simulink model "FaultModel (1)"  (R2018b)
settings: Solver=VariableStepAuto  StartTime=0.0  StopTime=0.05  RelTol=1e-3
undefined symbols (not defined in the file or in its folder): D1, Delta
libraries: powerlib x316
(part 1 of 4)
settings Model: Creator=DELL  LastModifiedBy=DELL
settings DataIOCC: ReturnWorkspaceOutputs=on
settings DebuggingCC: UnconnectedInputMsg=none  UnconnectedOutputMsg=none  UnconnectedLineMsg=none  SFMachineParentedDataDiag=error
settings ModelReferenceCC: EnableRefExpFcnMdlSchedulingChecks=off
settings RTWCC: Description=Generic Real-Time Target

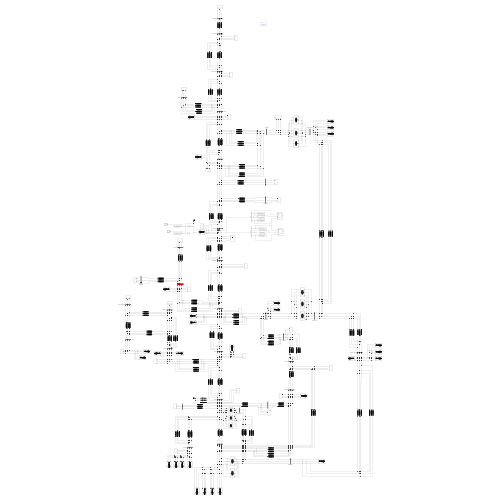
[thumbnail: Simulink's stored preview of the top-level diagram]
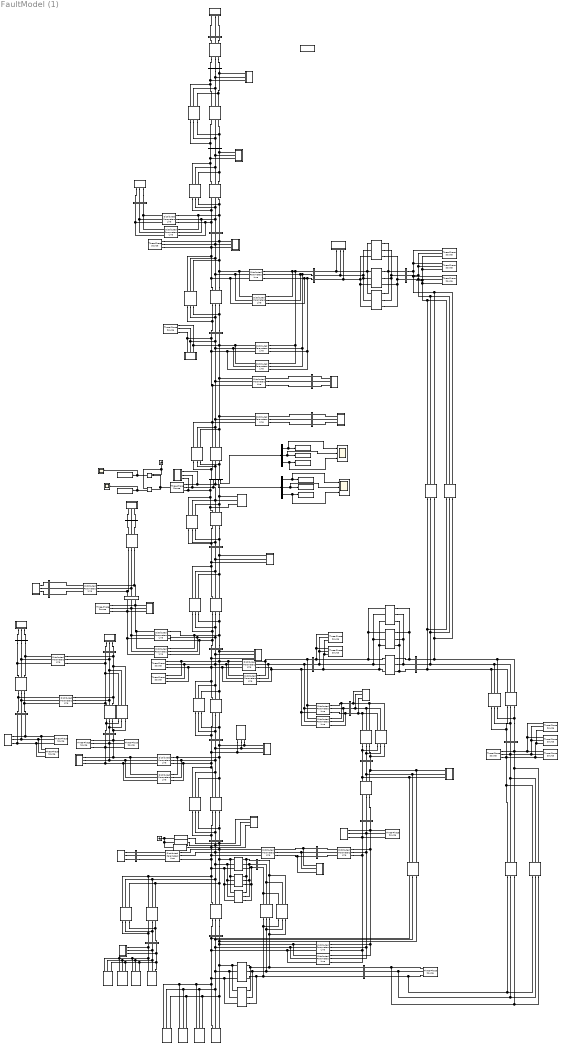
== system FaultModel (1) ==
  Amnura : powerlib/Measurements/Three-Phase V-I Measurement  VoltageMeasurement=no  SetLabelV=off  LabelV=Vabc  Vpu=off  VpuLL=off  CurrentMeasurement=no  SetLabelI=off  LabelI=Iabc  Ipu=off  Pbase=100e6  Vbase=500e3  OutputType=Complex  PhasorSimulation=off  PSBequivalent=0
  Baghabari : powerlib/Measurements/Three-Phase V-I Measurement  VoltageMeasurement=no  SetLabelV=off  LabelV=Vabc  Vpu=off  VpuLL=off  CurrentMeasurement=no  SetLabelI=off  LabelI=Iabc  Ipu=off  Pbase=100e6  Vbase=500e3  OutputType=Complex  PhasorSimulation=off  PSBequivalent=0
  Baghabari PP : powerlib/Measurements/Three-Phase V-I Measurement  VoltageMeasurement=no  SetLabelV=off  LabelV=Vabc  Vpu=off  VpuLL=off  CurrentMeasurement=no  SetLabelI=off  LabelI=Iabc  Ipu=off  Pbase=100e6  Vbase=500e3  OutputType=Complex  PhasorSimulation=off  PSBequivalent=0
  Barapukuria : powerlib/Measurements/Three-Phase V-I Measurement  VoltageMeasurement=no  SetLabelV=off  LabelV=Vabc  Vpu=off  VpuLL=off  CurrentMeasurement=no  SetLabelI=off  LabelI=Iabc  Ipu=off  Pbase=100e6  Vbase=500e3  OutputType=Complex  PhasorSimulation=off  PSBequivalent=0
  Barapukuria PP : powerlib/Measurements/Three-Phase V-I Measurement  VoltageMeasurement=no  SetLabelV=off  LabelV=Vabc  Vpu=off  VpuLL=off  CurrentMeasurement=no  SetLabelI=off  LabelI=Iabc  Ipu=off  Pbase=100e6  Vbase=500e3  OutputType=Complex  PhasorSimulation=off  PSBequivalent=0
  Bheramara : powerlib/Measurements/Three-Phase V-I Measurement  VoltageMeasurement=no  SetLabelV=off  LabelV=Vabc  Vpu=off  VpuLL=off  CurrentMeasurement=no  SetLabelI=off  LabelI=Iabc  Ipu=off  Pbase=100e6  Vbase=500e3  OutputType=Complex  PhasorSimulation=off  PSBequivalent=0
  Bogura : powerlib/Measurements/Three-Phase V-I Measurement  VoltageMeasurement=no  SetLabelV=off  LabelV=Vabc  Vpu=off  VpuLL=off  CurrentMeasurement=no  SetLabelI=off  LabelI=Iabc  Ipu=off  Pbase=100e6  Vbase=500e3  OutputType=Complex  PhasorSimulation=off  PSBequivalent=0
  Bogura New : powerlib/Measurements/Three-Phase V-I Measurement  VoltageMeasurement=no  SetLabelV=off  LabelV=Vabc  Vpu=off  VpuLL=off  CurrentMeasurement=no  SetLabelI=off  LabelI=Iabc  Ipu=off  Pbase=100e6  Vbase=500e3  OutputType=Complex  PhasorSimulation=off  PSBequivalent=0
  Bogura New PP : powerlib/Measurements/Three-Phase V-I Measurement  VoltageMeasurement=no  SetLabelV=off  LabelV=Vabc  Vpu=off  VpuLL=off  CurrentMeasurement=no  SetLabelI=off  LabelI=Iabc  Ipu=off  Pbase=100e6  Vbase=500e3  OutputType=Complex  PhasorSimulation=off  PSBequivalent=0
  Chapai Nawabganj : powerlib/Measurements/Three-Phase V-I Measurement  VoltageMeasurement=no  SetLabelV=off  LabelV=Vabc  Vpu=off  VpuLL=off  CurrentMeasurement=no  SetLabelI=off  LabelI=Iabc  Ipu=off  Pbase=100e6  Vbase=500e3  OutputType=Complex  PhasorSimulation=off  PSBequivalent=0
  Current Measurement : powerlib/Measurements/Current Measurement  PhasorSimulation=off  OutputType=Complex  PSBequivalent=0
  Demux : Demux  Outputs=3
  Demux1 : Demux  Outputs=3
  Distributed Parameters Line : powerlib/Elements/Distributed Parameters Line  Phases=3  Length=45  Frequency=50  Resistance=[0.01273 0.3864]  Inductance="[0.9337e-3  4.1264e-3]"  Capacitance=[12.74e-9 7.751e-9]  x1=[0 0 0 0; 0.0001244 0 0 0; 0.0002488 0 0 0; 0.0003733 0 0 0; 0.0004977 0 0 0; 0.0006221 0 0 0]  x2=[0 0 0 0; 0.0001244 0 0 0; 0.0002488 0 0 0; 0.0003733 0 0 0; 0.0004977 0 0 0; 0.0006221 0 0 0]  x3=[0 0 0 0; 0.0001244 0 0 0; 0.0002488 0 0 0; 0.0003733 0 0 0; 0.0004977 0 0 0; 0.0006221 0 0 0]  x4=[0 0 0 0; 0.0001244 0 0 0; 0.0002488 0 0 0; 0.0003733 0 0 0; 0.0004977 0 0 0; 0.0006221 0 0 0]  x5=0  V1=ones(3,3)  V2=ones(3,3)  I1=ones(3,3)  I2=ones(3,3)  nHarmo=1  Measurements=None  Decoupling=off  VsMag0=0  VrMag0=0  VsAngle0=0  VrAngle0=0  IsMag0=0  IrMag0=0  IsAngle0=0  IrAngle0=0
  Distributed Parameters Line1 : powerlib/Elements/Distributed Parameters Line  Phases=3  Length=45  Frequency=50  Resistance=[0.01273 0.3864]  Inductance="[0.9337e-3  4.1264e-3]"  Capacitance=[12.74e-9 7.751e-9]  x1=[0 0 0 0; 0.0001244 0 0 0; 0.0002488 0 0 0; 0.0003733 0 0 0; 0.0004977 0 0 0; 0.0006221 0 0 0]  x2=[0 0 0 0; 0.0001244 0 0 0; 0.0002488 0 0 0; 0.0003733 0 0 0; 0.0004977 0 0 0; 0.0006221 0 0 0]  x3=[0 0 0 0; 0.0001244 0 0 0; 0.0002488 0 0 0; 0.0003733 0 0 0; 0.0004977 0 0 0; 0.0006221 0 0 0]  x4=[0 0 0 0; 0.0001244 0 0 0; 0.0002488 0 0 0; 0.0003733 0 0 0; 0.0004977 0 0 0; 0.0006221 0 0 0]  x5=0  V1=ones(3,3)  V2=ones(3,3)  I1=ones(3,3)  I2=ones(3,3)  nHarmo=1  Measurements=None  Decoupling=off  VsMag0=0  VrMag0=0  VsAngle0=0  VrAngle0=0  IsMag0=0  IrMag0=0  IsAngle0=0  IrAngle0=0
  Distributed Parameters Line{9..10,44..45} (4 alike) : powerlib/Elements/Distributed Parameters Line  Phases=3  Length=36  Frequency=50  Resistance=[0.01273 0.3864]  Inductance="[0.9337e-3  4.1264e-3]"  Capacitance=[12.74e-9 7.751e-9]  x1=[0 0 0 0; 0.0001244 0 0 0; 0.0002488 0 0 0; 0.0003733 0 0 0; 0.0004977 0 0 0; 0.0006221 0 0 0]  x2=[0 0 0 0; 0.0001244 0 0 0; 0.0002488 0 0 0; 0.0003733 0 0 0; 0.0004977 0 0 0; 0.0006221 0 0 0]  x3=[0 0 0 0; 0.0001244 0 0 0; 0.0002488 0 0 0; 0.0003733 0 0 0; 0.0004977 0 0 0; 0.0006221 0 0 0]  x4=[0 0 0 0; 0.0001244 0 0 0; 0.0002488 0 0 0; 0.0003733 0 0 0; 0.0004977 0 0 0; 0.0006221 0 0 0]  x5=0  V1=ones(3,3)  V2=ones(3,3)  I1=ones(3,3)  I2=ones(3,3)  nHarmo=1  Measurements=None  Decoupling=off  VsMag0=0  VrMag0=0  VsAngle0=0  VrAngle0=0  IsMag0=0  IrMag0=0  IsAngle0=0  IrAngle0=0
  Distributed Parameters Line{11..12,29..30} (4 alike) : powerlib/Elements/Distributed Parameters Line  Phases=3  Length=42  Frequency=50  Resistance=[0.01273 0.3864]  Inductance="[0.9337e-3  4.1264e-3]"  Capacitance=[12.74e-9 7.751e-9]  x1=[0 0 0 0; 0.0001244 0 0 0; 0.0002488 0 0 0; 0.0003733 0 0 0; 0.0004977 0 0 0; 0.0006221 0 0 0]  x2=[0 0 0 0; 0.0001244 0 0 0; 0.0002488 0 0 0; 0.0003733 0 0 0; 0.0004977 0 0 0; 0.0006221 0 0 0]  x3=[0 0 0 0; 0.0001244 0 0 0; 0.0002488 0 0 0; 0.0003733 0 0 0; 0.0004977 0 0 0; 0.0006221 0 0 0]  x4=[0 0 0 0; 0.0001244 0 0 0; 0.0002488 0 0 0; 0.0003733 0 0 0; 0.0004977 0 0 0; 0.0006221 0 0 0]  x5=0  V1=ones(3,3)  V2=ones(3,3)  I1=ones(3,3)  I2=ones(3,3)  nHarmo=1  Measurements=None  Decoupling=off  VsMag0=0  VrMag0=0  VsAngle0=0  VrAngle0=0  IsMag0=0  IrMag0=0  IsAngle0=0  IrAngle0=0
  Distributed Parameters Line13 : powerlib/Elements/Distributed Parameters Line  Phases=3  Length=40.95  Frequency=50  Resistance=[0.01273 0.3864]  Inductance="[0.9337e-3  4.1264e-3]"  Capacitance=[12.74e-9 7.751e-9]  x1=[0 0 0 0; 0.0001244 0 0 0; 0.0002488 0 0 0; 0.0003733 0 0 0; 0.0004977 0 0 0; 0.0006221 0 0 0]  x2=[0 0 0 0; 0.0001244 0 0 0; 0.0002488 0 0 0; 0.0003733 0 0 0; 0.0004977 0 0 0; 0.0006221 0 0 0]  x3=[0 0 0 0; 0.0001244 0 0 0; 0.0002488 0 0 0; 0.0003733 0 0 0; 0.0004977 0 0 0; 0.0006221 0 0 0]  x4=[0 0 0 0; 0.0001244 0 0 0; 0.0002488 0 0 0; 0.0003733 0 0 0; 0.0004977 0 0 0; 0.0006221 0 0 0]  x5=0  V1=ones(3,3)  V2=ones(3,3)  I1=ones(3,3)  I2=ones(3,3)  nHarmo=1  Measurements=None  Decoupling=off  VsMag0=0  VrMag0=0  VsAngle0=0  VrAngle0=0  IsMag0=0  IrMag0=0  IsAngle0=0  IrAngle0=0
  Distributed Parameters Line14 : powerlib/Elements/Distributed Parameters Line  Phases=3  Length=38  Frequency=50  Resistance=[0.01273 0.3864]  Inductance="[0.9337e-3  4.1264e-3]"  Capacitance=[12.74e-9 7.751e-9]  x1=[0 0 0 0; 0.0001244 0 0 0; 0.0002488 0 0 0; 0.0003733 0 0 0; 0.0004977 0 0 0; 0.0006221 0 0 0]  x2=[0 0 0 0; 0.0001244 0 0 0; 0.0002488 0 0 0; 0.0003733 0 0 0; 0.0004977 0 0 0; 0.0006221 0 0 0]  x3=[0 0 0 0; 0.0001244 0 0 0; 0.0002488 0 0 0; 0.0003733 0 0 0; 0.0004977 0 0 0; 0.0006221 0 0 0]  x4=[0 0 0 0; 0.0001244 0 0 0; 0.0002488 0 0 0; 0.0003733 0 0 0; 0.0004977 0 0 0; 0.0006221 0 0 0]  x5=0  V1=ones(3,3)  V2=ones(3,3)  I1=ones(3,3)  I2=ones(3,3)  nHarmo=1  Measurements=None  Decoupling=off  VsMag0=0  VrMag0=0  VsAngle0=0  VrAngle0=0  IsMag0=0  IrMag0=0  IsAngle0=0  IrAngle0=0
  Distributed Parameters Line15 : powerlib/Elements/Distributed Parameters Line  Phases=3  Length=52  Frequency=50  Resistance=[0.01273 0.3864]  Inductance="[0.9337e-3  4.1264e-3]"  Capacitance=[12.74e-9 7.751e-9]  x1=[0 0 0 0; 0.0001244 0 0 0; 0.0002488 0 0 0; 0.0003733 0 0 0; 0.0004977 0 0 0; 0.0006221 0 0 0]  x2=[0 0 0 0; 0.0001244 0 0 0; 0.0002488 0 0 0; 0.0003733 0 0 0; 0.0004977 0 0 0; 0.0006221 0 0 0]  x3=[0 0 0 0; 0.0001244 0 0 0; 0.0002488 0 0 0; 0.0003733 0 0 0; 0.0004977 0 0 0; 0.0006221 0 0 0]  x4=[0 0 0 0; 0.0001244 0 0 0; 0.0002488 0 0 0; 0.0003733 0 0 0; 0.0004977 0 0 0; 0.0006221 0 0 0]  x5=0  V1=ones(3,3)  V2=ones(3,3)  I1=ones(3,3)  I2=ones(3,3)  nHarmo=1  Measurements=None  Decoupling=off  VsMag0=0  VrMag0=0  VsAngle0=0  VrAngle0=0  IsMag0=0  IrMag0=0  IsAngle0=0  IrAngle0=0
  Distributed Parameters Line16 : powerlib/Elements/Distributed Parameters Line  Phases=3  Length=52  Frequency=50  Resistance=[0.01273 0.3864]  Inductance="[0.9337e-3  4.1264e-3]"  Capacitance=[12.74e-9 7.751e-9]  x1=[0 0 0 0; 0.0001244 0 0 0; 0.0002488 0 0 0; 0.0003733 0 0 0; 0.0004977 0 0 0; 0.0006221 0 0 0]  x2=[0 0 0 0; 0.0001244 0 0 0; 0.0002488 0 0 0; 0.0003733 0 0 0; 0.0004977 0 0 0; 0.0006221 0 0 0]  x3=[0 0 0 0; 0.0001244 0 0 0; 0.0002488 0 0 0; 0.0003733 0 0 0; 0.0004977 0 0 0; 0.0006221 0 0 0]  x4=[0 0 0 0; 0.0001244 0 0 0; 0.0002488 0 0 0; 0.0003733 0 0 0; 0.0004977 0 0 0; 0.0006221 0 0 0]  x5=0  V1=ones(3,3)  V2=ones(3,3)  I1=ones(3,3)  I2=ones(3,3)  nHarmo=1  Measurements=None  Decoupling=off  VsMag0=0  VrMag0=0  VsAngle0=0  VrAngle0=0  IsMag0=0  IrMag0=0  IsAngle0=0  IrAngle0=0
  Distributed Parameters Line17 : powerlib/Elements/Distributed Parameters Line  Phases=3  Length=0.7  Frequency=50  Resistance=[0.01273 0.3864]  Inductance="[0.9337e-3  4.1264e-3]"  Capacitance=[12.74e-9 7.751e-9]  x1=[0 0 0 0; 0.0001244 0 0 0; 0.0002488 0 0 0; 0.0003733 0 0 0; 0.0004977 0 0 0; 0.0006221 0 0 0]  x2=[0 0 0 0; 0.0001244 0 0 0; 0.0002488 0 0 0; 0.0003733 0 0 0; 0.0004977 0 0 0; 0.0006221 0 0 0]  x3=[0 0 0 0; 0.0001244 0 0 0; 0.0002488 0 0 0; 0.0003733 0 0 0; 0.0004977 0 0 0; 0.0006221 0 0 0]  x4=[0 0 0 0; 0.0001244 0 0 0; 0.0002488 0 0 0; 0.0003733 0 0 0; 0.0004977 0 0 0; 0.0006221 0 0 0]  x5=0  V1=ones(3,3)  V2=ones(3,3)  I1=ones(3,3)  I2=ones(3,3)  nHarmo=1  Measurements=None  Decoupling=off  VsMag0=0  VrMag0=0  VsAngle0=0  VrAngle0=0  IsMag0=0  IrMag0=0  IsAngle0=0  IrAngle0=0
  Distributed Parameters Line18 : powerlib/Elements/Distributed Parameters Line  Phases=3  Length=0.7  Frequency=50  Resistance=[0.01273 0.3864]  Inductance="[0.9337e-3  4.1264e-3]"  Capacitance=[12.74e-9 7.751e-9]  x1=[0 0 0 0; 0.0001244 0 0 0; 0.0002488 0 0 0; 0.0003733 0 0 0; 0.0004977 0 0 0; 0.0006221 0 0 0]  x2=[0 0 0 0; 0.0001244 0 0 0; 0.0002488 0 0 0; 0.0003733 0 0 0; 0.0004977 0 0 0; 0.0006221 0 0 0]  x3=[0 0 0 0; 0.0001244 0 0 0; 0.0002488 0 0 0; 0.0003733 0 0 0; 0.0004977 0 0 0; 0.0006221 0 0 0]  x4=[0 0 0 0; 0.0001244 0 0 0; 0.0002488 0 0 0; 0.0003733 0 0 0; 0.0004977 0 0 0; 0.0006221 0 0 0]  x5=0  V1=ones(3,3)  V2=ones(3,3)  I1=ones(3,3)  I2=ones(3,3)  nHarmo=1  Measurements=None  Decoupling=off  VsMag0=0  VrMag0=0  VsAngle0=0  VrAngle0=0  IsMag0=0  IrMag0=0  IsAngle0=0  IrAngle0=0
  Distributed Parameters Line19 : powerlib/Elements/Distributed Parameters Line  Phases=3  Length=50  Frequency=50  Resistance=[0.01273 0.3864]  Inductance="[0.9337e-3  4.1264e-3]"  Capacitance=[12.74e-9 7.751e-9]  x1=[0 0 0 0; 0.0001244 0 0 0; 0.0002488 0 0 0; 0.0003733 0 0 0; 0.0004977 0 0 0; 0.0006221 0 0 0]  x2=[0 0 0 0; 0.0001244 0 0 0; 0.0002488 0 0 0; 0.0003733 0 0 0; 0.0004977 0 0 0; 0.0006221 0 0 0]  x3=[0 0 0 0; 0.0001244 0 0 0; 0.0002488 0 0 0; 0.0003733 0 0 0; 0.0004977 0 0 0; 0.0006221 0 0 0]  x4=[0 0 0 0; 0.0001244 0 0 0; 0.0002488 0 0 0; 0.0003733 0 0 0; 0.0004977 0 0 0; 0.0006221 0 0 0]  x5=0  V1=ones(3,3)  V2=ones(3,3)  I1=ones(3,3)  I2=ones(3,3)  nHarmo=1  Measurements=None  Decoupling=off  VsMag0=0  VrMag0=0  VsAngle0=0  VrAngle0=0  IsMag0=0  IrMag0=0  IsAngle0=0  IrAngle0=0
  Distributed Parameters Line2 : powerlib/Elements/Distributed Parameters Line  Phases=3  Length=45  Frequency=50  Resistance=[0.01273 0.3864]  Inductance="[0.9337e-3  4.1264e-3]"  Capacitance=[12.74e-9 7.751e-9]  x1=[0 0 0 0; 0.0001244 0 0 0; 0.0002488 0 0 0; 0.0003733 0 0 0; 0.0004977 0 0 0; 0.0006221 0 0 0]  x2=[0 0 0 0; 0.0001244 0 0 0; 0.0002488 0 0 0; 0.0003733 0 0 0; 0.0004977 0 0 0; 0.0006221 0 0 0]  x3=[0 0 0 0; 0.0001244 0 0 0; 0.0002488 0 0 0; 0.0003733 0 0 0; 0.0004977 0 0 0; 0.0006221 0 0 0]  x4=[0 0 0 0; 0.0001244 0 0 0; 0.0002488 0 0 0; 0.0003733 0 0 0; 0.0004977 0 0 0; 0.0006221 0 0 0]  x5=0  V1=ones(3,3)  V2=ones(3,3)  I1=ones(3,3)  I2=ones(3,3)  nHarmo=1  Measurements=None  Decoupling=off  VsMag0=0  VrMag0=0  VsAngle0=0  VrAngle0=0  IsMag0=0  IrMag0=0  IsAngle0=0  IrAngle0=0
  Distributed Parameters Line20 : powerlib/Elements/Distributed Parameters Line  Phases=3  Length=50  Frequency=50  Resistance=[0.01273 0.3864]  Inductance="[0.9337e-3  4.1264e-3]"  Capacitance=[12.74e-9 7.751e-9]  x1=[0 0 0 0; 0.0001244 0 0 0; 0.0002488 0 0 0; 0.0003733 0 0 0; 0.0004977 0 0 0; 0.0006221 0 0 0]  x2=[0 0 0 0; 0.0001244 0 0 0; 0.0002488 0 0 0; 0.0003733 0 0 0; 0.0004977 0 0 0; 0.0006221 0 0 0]  x3=[0 0 0 0; 0.0001244 0 0 0; 0.0002488 0 0 0; 0.0003733 0 0 0; 0.0004977 0 0 0; 0.0006221 0 0 0]  x4=[0 0 0 0; 0.0001244 0 0 0; 0.0002488 0 0 0; 0.0003733 0 0 0; 0.0004977 0 0 0; 0.0006221 0 0 0]  x5=0  V1=ones(3,3)  V2=ones(3,3)  I1=ones(3,3)  I2=ones(3,3)  nHarmo=1  Measurements=None  Decoupling=off  VsMag0=0  VrMag0=0  VsAngle0=0  VrAngle0=0  IsMag0=0  IrMag0=0  IsAngle0=0  IrAngle0=0
  Distributed Parameters Line21 : powerlib/Elements/Distributed Parameters Line  Phases=3  Length=44  Frequency=50  Resistance=[0.01273 0.3864]  Inductance="[0.9337e-3  4.1264e-3]"  Capacitance=[12.74e-9 7.751e-9]  x1=[0 0 0 0; 0.0001244 0 0 0; 0.0002488 0 0 0; 0.0003733 0 0 0; 0.0004977 0 0 0; 0.0006221 0 0 0]  x2=[0 0 0 0; 0.0001244 0 0 0; 0.0002488 0 0 0; 0.0003733 0 0 0; 0.0004977 0 0 0; 0.0006221 0 0 0]  x3=[0 0 0 0; 0.0001244 0 0 0; 0.0002488 0 0 0; 0.0003733 0 0 0; 0.0004977 0 0 0; 0.0006221 0 0 0]  x4=[0 0 0 0; 0.0001244 0 0 0; 0.0002488 0 0 0; 0.0003733 0 0 0; 0.0004977 0 0 0; 0.0006221 0 0 0]  x5=0  V1=ones(3,3)  V2=ones(3,3)  I1=ones(3,3)  I2=ones(3,3)  nHarmo=1  Measurements=None  Decoupling=off  VsMag0=0  VrMag0=0  VsAngle0=0  VrAngle0=0  IsMag0=0  IrMag0=0  IsAngle0=0  IrAngle0=0
  Distributed Parameters Line22 : powerlib/Elements/Distributed Parameters Line  Phases=3  Length=44  Frequency=50  Resistance=[0.01273 0.3864]  Inductance="[0.9337e-3  4.1264e-3]"  Capacitance=[12.74e-9 7.751e-9]  x1=[0 0 0 0; 0.0001244 0 0 0; 0.0002488 0 0 0; 0.0003733 0 0 0; 0.0004977 0 0 0; 0.0006221 0 0 0]  x2=[0 0 0 0; 0.0001244 0 0 0; 0.0002488 0 0 0; 0.0003733 0 0 0; 0.0004977 0 0 0; 0.0006221 0 0 0]  x3=[0 0 0 0; 0.0001244 0 0 0; 0.0002488 0 0 0; 0.0003733 0 0 0; 0.0004977 0 0 0; 0.0006221 0 0 0]  x4=[0 0 0 0; 0.0001244 0 0 0; 0.0002488 0 0 0; 0.0003733 0 0 0; 0.0004977 0 0 0; 0.0006221 0 0 0]  x5=0  V1=ones(3,3)  V2=ones(3,3)  I1=ones(3,3)  I2=ones(3,3)  nHarmo=1  Measurements=None  Decoupling=off  VsMag0=0  VrMag0=0  VsAngle0=0  VrAngle0=0  IsMag0=0  IrMag0=0  IsAngle0=0  IrAngle0=0
  Distributed Parameters Line23 : powerlib/Elements/Distributed Parameters Line  Phases=3  Length=46.2  Frequency=50  Resistance=[0.01273 0.3864]  Inductance="[0.9337e-3  4.1264e-3]"  Capacitance=[12.74e-9 7.751e-9]  x1=[0 0 0 0; 0.0001244 0 0 0; 0.0002488 0 0 0; 0.0003733 0 0 0; 0.0004977 0 0 0; 0.0006221 0 0 0]  x2=[0 0 0 0; 0.0001244 0 0 0; 0.0002488 0 0 0; 0.0003733 0 0 0; 0.0004977 0 0 0; 0.0006221 0 0 0]  x3=[0 0 0 0; 0.0001244 0 0 0; 0.0002488 0 0 0; 0.0003733 0 0 0; 0.0004977 0 0 0; 0.0006221 0 0 0]  x4=[0 0 0 0; 0.0001244 0 0 0; 0.0002488 0 0 0; 0.0003733 0 0 0; 0.0004977 0 0 0; 0.0006221 0 0 0]  x5=0  V1=ones(3,3)  V2=ones(3,3)  I1=ones(3,3)  I2=ones(3,3)  nHarmo=1  Measurements=None  Decoupling=off  VsMag0=0  VrMag0=0  VsAngle0=0  VrAngle0=0  IsMag0=0  IrMag0=0  IsAngle0=0  IrAngle0=0
  Distributed Parameters Line24 : powerlib/Elements/Distributed Parameters Line  Phases=3  Length=46  Frequency=50  Resistance=[0.01273 0.3864]  Inductance="[0.9337e-3  4.1264e-3]"  Capacitance=[12.74e-9 7.751e-9]  x1=[0 0 0 0; 0.0001244 0 0 0; 0.0002488 0 0 0; 0.0003733 0 0 0; 0.0004977 0 0 0; 0.0006221 0 0 0]  x2=[0 0 0 0; 0.0001244 0 0 0; 0.0002488 0 0 0; 0.0003733 0 0 0; 0.0004977 0 0 0; 0.0006221 0 0 0]  x3=[0 0 0 0; 0.0001244 0 0 0; 0.0002488 0 0 0; 0.0003733 0 0 0; 0.0004977 0 0 0; 0.0006221 0 0 0]  x4=[0 0 0 0; 0.0001244 0 0 0; 0.0002488 0 0 0; 0.0003733 0 0 0; 0.0004977 0 0 0; 0.0006221 0 0 0]  x5=0  V1=ones(3,3)  V2=ones(3,3)  I1=ones(3,3)  I2=ones(3,3)  nHarmo=1  Measurements=None  Decoupling=off  VsMag0=0  VrMag0=0  VsAngle0=0  VrAngle0=0  IsMag0=0  IrMag0=0  IsAngle0=0  IrAngle0=0
  Distributed Parameters Line25 : powerlib/Elements/Distributed Parameters Line  Phases=3  Length=1.5  Frequency=50  Resistance=[0.01273 0.3864]  Inductance="[0.9337e-3  4.1264e-3]"  Capacitance=[12.74e-9 7.751e-9]  x1=[0 0 0 0; 0.0001244 0 0 0; 0.0002488 0 0 0; 0.0003733 0 0 0; 0.0004977 0 0 0; 0.0006221 0 0 0]  x2=[0 0 0 0; 0.0001244 0 0 0; 0.0002488 0 0 0; 0.0003733 0 0 0; 0.0004977 0 0 0; 0.0006221 0 0 0]  x3=[0 0 0 0; 0.0001244 0 0 0; 0.0002488 0 0 0; 0.0003733 0 0 0; 0.0004977 0 0 0; 0.0006221 0 0 0]  x4=[0 0 0 0; 0.0001244 0 0 0; 0.0002488 0 0 0; 0.0003733 0 0 0; 0.0004977 0 0 0; 0.0006221 0 0 0]  x5=0  V1=ones(3,3)  V2=ones(3,3)  I1=ones(3,3)  I2=ones(3,3)  nHarmo=1  Measurements=None  Decoupling=off  VsMag0=0  VrMag0=0  VsAngle0=0  VrAngle0=0  IsMag0=0  IrMag0=0  IsAngle0=0  IrAngle0=0
  Distributed Parameters Line26 : powerlib/Elements/Distributed Parameters Line  Phases=3  Length=1.5  Frequency=50  Resistance=[0.01273 0.3864]  Inductance="[0.9337e-3  4.1264e-3]"  Capacitance=[12.74e-9 7.751e-9]  x1=[0 0 0 0; 0.0001244 0 0 0; 0.0002488 0 0 0; 0.0003733 0 0 0; 0.0004977 0 0 0; 0.0006221 0 0 0]  x2=[0 0 0 0; 0.0001244 0 0 0; 0.0002488 0 0 0; 0.0003733 0 0 0; 0.0004977 0 0 0; 0.0006221 0 0 0]  x3=[0 0 0 0; 0.0001244 0 0 0; 0.0002488 0 0 0; 0.0003733 0 0 0; 0.0004977 0 0 0; 0.0006221 0 0 0]  x4=[0 0 0 0; 0.0001244 0 0 0; 0.0002488 0 0 0; 0.0003733 0 0 0; 0.0004977 0 0 0; 0.0006221 0 0 0]  x5=0  V1=ones(3,3)  V2=ones(3,3)  I1=ones(3,3)  I2=ones(3,3)  nHarmo=1  Measurements=None  Decoupling=off  VsMag0=0  VrMag0=0  VsAngle0=0  VrAngle0=0  IsMag0=0  IrMag0=0  IsAngle0=0  IrAngle0=0
  Distributed Parameters Line27 : powerlib/Elements/Distributed Parameters Line  Phases=3  Length=61  Frequency=50  Resistance=[0.01273 0.3864]  Inductance="[0.9337e-3  4.1264e-3]"  Capacitance=[12.74e-9 7.751e-9]  x1=[0 0 0 0; 0.0001244 0 0 0; 0.0002488 0 0 0; 0.0003733 0 0 0; 0.0004977 0 0 0; 0.0006221 0 0 0]  x2=[0 0 0 0; 0.0001244 0 0 0; 0.0002488 0 0 0; 0.0003733 0 0 0; 0.0004977 0 0 0; 0.0006221 0 0 0]  x3=[0 0 0 0; 0.0001244 0 0 0; 0.0002488 0 0 0; 0.0003733 0 0 0; 0.0004977 0 0 0; 0.0006221 0 0 0]  x4=[0 0 0 0; 0.0001244 0 0 0; 0.0002488 0 0 0; 0.0003733 0 0 0; 0.0004977 0 0 0; 0.0006221 0 0 0]  x5=0  V1=ones(3,3)  V2=ones(3,3)  I1=ones(3,3)  I2=ones(3,3)  nHarmo=1  Measurements=None  Decoupling=off  VsMag0=0  VrMag0=0  VsAngle0=0  VrAngle0=0  IsMag0=0  IrMag0=0  IsAngle0=0  IrAngle0=0
  Distributed Parameters Line28 : powerlib/Elements/Distributed Parameters Line  Phases=3  Length=61  Frequency=50  Resistance=[0.01273 0.3864]  Inductance="[0.9337e-3  4.1264e-3]"  Capacitance=[12.74e-9 7.751e-9]  x1=[0 0 0 0; 0.0001244 0 0 0; 0.0002488 0 0 0; 0.0003733 0 0 0; 0.0004977 0 0 0; 0.0006221 0 0 0]  x2=[0 0 0 0; 0.0001244 0 0 0; 0.0002488 0 0 0; 0.0003733 0 0 0; 0.0004977 0 0 0; 0.0006221 0 0 0]  x3=[0 0 0 0; 0.0001244 0 0 0; 0.0002488 0 0 0; 0.0003733 0 0 0; 0.0004977 0 0 0; 0.0006221 0 0 0]  x4=[0 0 0 0; 0.0001244 0 0 0; 0.0002488 0 0 0; 0.0003733 0 0 0; 0.0004977 0 0 0; 0.0006221 0 0 0]  x5=0  V1=ones(3,3)  V2=ones(3,3)  I1=ones(3,3)  I2=ones(3,3)  nHarmo=1  Measurements=None  Decoupling=off  VsMag0=0  VrMag0=0  VsAngle0=0  VrAngle0=0  IsMag0=0  IrMag0=0  IsAngle0=0  IrAngle0=0
  Distributed Parameters Line3 : powerlib/Elements/Distributed Parameters Line  Phases=3  Length=24.5  Frequency=50  Resistance=[0.01273 0.3864]  Inductance="[0.9337e-3  4.1264e-3]"  Capacitance=[12.74e-9 7.751e-9]  x1=[0 0 0 0; 0.0001244 0 0 0; 0.0002488 0 0 0; 0.0003733 0 0 0; 0.0004977 0 0 0; 0.0006221 0 0 0]  x2=[0 0 0 0; 0.0001244 0 0 0; 0.0002488 0 0 0; 0.0003733 0 0 0; 0.0004977 0 0 0; 0.0006221 0 0 0]  x3=[0 0 0 0; 0.0001244 0 0 0; 0.0002488 0 0 0; 0.0003733 0 0 0; 0.0004977 0 0 0; 0.0006221 0 0 0]  x4=[0 0 0 0; 0.0001244 0 0 0; 0.0002488 0 0 0; 0.0003733 0 0 0; 0.0004977 0 0 0; 0.0006221 0 0 0]  x5=0  V1=ones(3,3)  V2=ones(3,3)  I1=ones(3,3)  I2=ones(3,3)  nHarmo=1  Measurements=None  Decoupling=off  VsMag0=0  VrMag0=0  VsAngle0=0  VrAngle0=0  IsMag0=0  IrMag0=0  IsAngle0=0  IrAngle0=0
  Distributed Parameters Line31 : powerlib/Elements/Distributed Parameters Line  Phases=3  Length=40  Frequency=50  Resistance=[0.01273 0.3864]  Inductance="[0.9337e-3  4.1264e-3]"  Capacitance=[12.74e-9 7.751e-9]  x1=[0 0 0 0; 0.0001244 0 0 0; 0.0002488 0 0 0; 0.0003733 0 0 0; 0.0004977 0 0 0; 0.0006221 0 0 0]  x2=[0 0 0 0; 0.0001244 0 0 0; 0.0002488 0 0 0; 0.0003733 0 0 0; 0.0004977 0 0 0; 0.0006221 0 0 0]  x3=[0 0 0 0; 0.0001244 0 0 0; 0.0002488 0 0 0; 0.0003733 0 0 0; 0.0004977 0 0 0; 0.0006221 0 0 0]  x4=[0 0 0 0; 0.0001244 0 0 0; 0.0002488 0 0 0; 0.0003733 0 0 0; 0.0004977 0 0 0; 0.0006221 0 0 0]  x5=0  V1=ones(3,3)  V2=ones(3,3)  I1=ones(3,3)  I2=ones(3,3)  nHarmo=1  Measurements=None  Decoupling=off  VsMag0=0  VrMag0=0  VsAngle0=0  VrAngle0=0  IsMag0=0  IrMag0=0  IsAngle0=0  IrAngle0=0
  Distributed Parameters Line32 : powerlib/Elements/Distributed Parameters Line  Phases=3  Length=37  Frequency=50  Resistance=[0.01273 0.3864]  Inductance="[0.9337e-3  4.1264e-3]"  Capacitance=[12.74e-9 7.751e-9]  x1=[0 0 0 0; 0.0001244 0 0 0; 0.0002488 0 0 0; 0.0003733 0 0 0; 0.0004977 0 0 0; 0.0006221 0 0 0]  x2=[0 0 0 0; 0.0001244 0 0 0; 0.0002488 0 0 0; 0.0003733 0 0 0; 0.0004977 0 0 0; 0.0006221 0 0 0]  x3=[0 0 0 0; 0.0001244 0 0 0; 0.0002488 0 0 0; 0.0003733 0 0 0; 0.0004977 0 0 0; 0.0006221 0 0 0]  x4=[0 0 0 0; 0.0001244 0 0 0; 0.0002488 0 0 0; 0.0003733 0 0 0; 0.0004977 0 0 0; 0.0006221 0 0 0]  x5=0  V1=ones(3,3)  V2=ones(3,3)  I1=ones(3,3)  I2=ones(3,3)  nHarmo=1  Measurements=None  Decoupling=off  VsMag0=0  VrMag0=0  VsAngle0=0  VrAngle0=0  IsMag0=0  IrMag0=0  IsAngle0=0  IrAngle0=0
  Distributed Parameters Line{7..8,33..34,42..43} (6 alike) : powerlib/Elements/Distributed Parameters Line  Phases=3  Length=30  Frequency=50  Resistance=[0.01273 0.3864]  Inductance="[0.9337e-3  4.1264e-3]"  Capacitance=[12.74e-9 7.751e-9]  x1=[0 0 0 0; 0.0001244 0 0 0; 0.0002488 0 0 0; 0.0003733 0 0 0; 0.0004977 0 0 0; 0.0006221 0 0 0]  x2=[0 0 0 0; 0.0001244 0 0 0; 0.0002488 0 0 0; 0.0003733 0 0 0; 0.0004977 0 0 0; 0.0006221 0 0 0]  x3=[0 0 0 0; 0.0001244 0 0 0; 0.0002488 0 0 0; 0.0003733 0 0 0; 0.0004977 0 0 0; 0.0006221 0 0 0]  x4=[0 0 0 0; 0.0001244 0 0 0; 0.0002488 0 0 0; 0.0003733 0 0 0; 0.0004977 0 0 0; 0.0006221 0 0 0]  x5=0  V1=ones(3,3)  V2=ones(3,3)  I1=ones(3,3)  I2=ones(3,3)  nHarmo=1  Measurements=None  Decoupling=off  VsMag0=0  VrMag0=0  VsAngle0=0  VrAngle0=0  IsMag0=0  IrMag0=0  IsAngle0=0  IrAngle0=0
  Distributed Parameters Line35 : powerlib/Elements/Distributed Parameters Line  Phases=3  Length=18  Frequency=50  Resistance=[0.01273 0.3864]  Inductance="[0.9337e-3  4.1264e-3]"  Capacitance=[12.74e-9 7.751e-9]  x1=[0 0 0 0; 0.0001244 0 0 0; 0.0002488 0 0 0; 0.0003733 0 0 0; 0.0004977 0 0 0; 0.0006221 0 0 0]  x2=[0 0 0 0; 0.0001244 0 0 0; 0.0002488 0 0 0; 0.0003733 0 0 0; 0.0004977 0 0 0; 0.0006221 0 0 0]  x3=[0 0 0 0; 0.0001244 0 0 0; 0.0002488 0 0 0; 0.0003733 0 0 0; 0.0004977 0 0 0; 0.0006221 0 0 0]  x4=[0 0 0 0; 0.0001244 0 0 0; 0.0002488 0 0 0; 0.0003733 0 0 0; 0.0004977 0 0 0; 0.0006221 0 0 0]  x5=0  V1=ones(3,3)  V2=ones(3,3)  I1=ones(3,3)  I2=ones(3,3)  nHarmo=1  Measurements=None  Decoupling=off  VsMag0=0  VrMag0=0  VsAngle0=0  VrAngle0=0  IsMag0=0  IrMag0=0  IsAngle0=0  IrAngle0=0
  Distributed Parameters Line36 : powerlib/Elements/Distributed Parameters Line  Phases=3  Length=5.4  Frequency=50  Resistance=[0.01273 0.3864]  Inductance="[0.9337e-3  4.1264e-3]"  Capacitance=[12.74e-9 7.751e-9]  x1=[0 0 0 0; 0.0001244 0 0 0; 0.0002488 0 0 0; 0.0003733 0 0 0; 0.0004977 0 0 0; 0.0006221 0 0 0]  x2=[0 0 0 0; 0.0001244 0 0 0; 0.0002488 0 0 0; 0.0003733 0 0 0; 0.0004977 0 0 0; 0.0006221 0 0 0]  x3=[0 0 0 0; 0.0001244 0 0 0; 0.0002488 0 0 0; 0.0003733 0 0 0; 0.0004977 0 0 0; 0.0006221 0 0 0]  x4=[0 0 0 0; 0.0001244 0 0 0; 0.0002488 0 0 0; 0.0003733 0 0 0; 0.0004977 0 0 0; 0.0006221 0 0 0]  x5=0  V1=ones(3,3)  V2=ones(3,3)  I1=ones(3,3)  I2=ones(3,3)  nHarmo=1  Measurements=None  Decoupling=off  VsMag0=0  VrMag0=0  VsAngle0=0  VrAngle0=0  IsMag0=0  IrMag0=0  IsAngle0=0  IrAngle0=0
  Distributed Parameters Line37 : powerlib/Elements/Distributed Parameters Line  Phases=3  Length=12.6  Frequency=50  Resistance=[0.01273 0.3864]  Inductance="[0.9337e-3  4.1264e-3]"  Capacitance=[12.74e-9 7.751e-9]  x1=[0 0 0 0; 0.0001244 0 0 0; 0.0002488 0 0 0; 0.0003733 0 0 0; 0.0004977 0 0 0; 0.0006221 0 0 0]  x2=[0 0 0 0; 0.0001244 0 0 0; 0.0002488 0 0 0; 0.0003733 0 0 0; 0.0004977 0 0 0; 0.0006221 0 0 0]  x3=[0 0 0 0; 0.0001244 0 0 0; 0.0002488 0 0 0; 0.0003733 0 0 0; 0.0004977 0 0 0; 0.0006221 0 0 0]  x4=[0 0 0 0; 0.0001244 0 0 0; 0.0002488 0 0 0; 0.0003733 0 0 0; 0.0004977 0 0 0; 0.0006221 0 0 0]  x5=0  V1=ones(3,3)  V2=ones(3,3)  I1=ones(3,3)  I2=ones(3,3)  nHarmo=1  Measurements=None  Decoupling=off  VsMag0=0  VrMag0=0  VsAngle0=0  VrAngle0=0  IsMag0=0  IrMag0=0  IsAngle0=0  IrAngle0=0
  Distributed Parameters Line38 : powerlib/Elements/Distributed Parameters Line  Phases=3  Length=7  Frequency=50  Resistance=[0.01273 0.3864]  Inductance="[0.9337e-3  4.1264e-3]"  Capacitance=[12.74e-9 7.751e-9]  x1=[0 0 0 0; 0.0001244 0 0 0; 0.0002488 0 0 0; 0.0003733 0 0 0; 0.0004977 0 0 0; 0.0006221 0 0 0]  x2=[0 0 0 0; 0.0001244 0 0 0; 0.0002488 0 0 0; 0.0003733 0 0 0; 0.0004977 0 0 0; 0.0006221 0 0 0]  x3=[0 0 0 0; 0.0001244 0 0 0; 0.0002488 0 0 0; 0.0003733 0 0 0; 0.0004977 0 0 0; 0.0006221 0 0 0]  x4=[0 0 0 0; 0.0001244 0 0 0; 0.0002488 0 0 0; 0.0003733 0 0 0; 0.0004977 0 0 0; 0.0006221 0 0 0]  x5=0  V1=ones(3,3)  V2=ones(3,3)  I1=ones(3,3)  I2=ones(3,3)  nHarmo=1  Measurements=None  Decoupling=off  VsMag0=0  VrMag0=0  VsAngle0=0  VrAngle0=0  IsMag0=0  IrMag0=0  IsAngle0=0  IrAngle0=0
  Distributed Parameters Line39 : powerlib/Elements/Distributed Parameters Line  Phases=3  Length=10  Frequency=50  Resistance=[0.01273 0.3864]  Inductance="[0.9337e-3  4.1264e-3]"  Capacitance=[12.74e-9 7.751e-9]  x1=[0 0 0 0; 0.0001244 0 0 0; 0.0002488 0 0 0; 0.0003733 0 0 0; 0.0004977 0 0 0; 0.0006221 0 0 0]  x2=[0 0 0 0; 0.0001244 0 0 0; 0.0002488 0 0 0; 0.0003733 0 0 0; 0.0004977 0 0 0; 0.0006221 0 0 0]  x3=[0 0 0 0; 0.0001244 0 0 0; 0.0002488 0 0 0; 0.0003733 0 0 0; 0.0004977 0 0 0; 0.0006221 0 0 0]  x4=[0 0 0 0; 0.0001244 0 0 0; 0.0002488 0 0 0; 0.0003733 0 0 0; 0.0004977 0 0 0; 0.0006221 0 0 0]  x5=0  V1=ones(3,3)  V2=ones(3,3)  I1=ones(3,3)  I2=ones(3,3)  nHarmo=1  Measurements=None  Decoupling=off  VsMag0=0  VrMag0=0  VsAngle0=0  VrAngle0=0  IsMag0=0  IrMag0=0  IsAngle0=0  IrAngle0=0
  Distributed Parameters Line4 : powerlib/Elements/Distributed Parameters Line  Phases=3  Length=24.5  Frequency=50  Resistance=[0.01273 0.3864]  Inductance="[0.9337e-3  4.1264e-3]"  Capacitance=[12.74e-9 7.751e-9]  x1=[0 0 0 0; 0.0001244 0 0 0; 0.0002488 0 0 0; 0.0003733 0 0 0; 0.0004977 0 0 0; 0.0006221 0 0 0]  x2=[0 0 0 0; 0.0001244 0 0 0; 0.0002488 0 0 0; 0.0003733 0 0 0; 0.0004977 0 0 0; 0.0006221 0 0 0]  x3=[0 0 0 0; 0.0001244 0 0 0; 0.0002488 0 0 0; 0.0003733 0 0 0; 0.0004977 0 0 0; 0.0006221 0 0 0]  x4=[0 0 0 0; 0.0001244 0 0 0; 0.0002488 0 0 0; 0.0003733 0 0 0; 0.0004977 0 0 0; 0.0006221 0 0 0]  x5=0  V1=ones(3,3)  V2=ones(3,3)  I1=ones(3,3)  I2=ones(3,3)  nHarmo=1  Measurements=None  Decoupling=off  VsMag0=0  VrMag0=0  VsAngle0=0  VrAngle0=0  IsMag0=0  IrMag0=0  IsAngle0=0  IrAngle0=0
  Distributed Parameters Line40 : powerlib/Elements/Distributed Parameters Line  Phases=3  Length=10  Frequency=50  Resistance=[0.01273 0.3864]  Inductance="[0.9337e-3  4.1264e-3]"  Capacitance=[12.74e-9 7.751e-9]  x1=[0 0 0 0; 0.0001244 0 0 0; 0.0002488 0 0 0; 0.0003733 0 0 0; 0.0004977 0 0 0; 0.0006221 0 0 0]  x2=[0 0 0 0; 0.0001244 0 0 0; 0.0002488 0 0 0; 0.0003733 0 0 0; 0.0004977 0 0 0; 0.0006221 0 0 0]  x3=[0 0 0 0; 0.0001244 0 0 0; 0.0002488 0 0 0; 0.0003733 0 0 0; 0.0004977 0 0 0; 0.0006221 0 0 0]  x4=[0 0 0 0; 0.0001244 0 0 0; 0.0002488 0 0 0; 0.0003733 0 0 0; 0.0004977 0 0 0; 0.0006221 0 0 0]  x5=0  V1=ones(3,3)  V2=ones(3,3)  I1=ones(3,3)  I2=ones(3,3)  nHarmo=1  Measurements=None  Decoupling=off  VsMag0=0  VrMag0=0  VsAngle0=0  VrAngle0=0  IsMag0=0  IrMag0=0  IsAngle0=0  IrAngle0=0
  Distributed Parameters Line41 : powerlib/Elements/Distributed Parameters Line  Phases=3  Length=63  Frequency=50  Resistance=[0.01273 0.3864]  Inductance="[0.9337e-3  4.1264e-3]"  Capacitance=[12.74e-9 7.751e-9]  x1=[0 0 0 0; 0.0001244 0 0 0; 0.0002488 0 0 0; 0.0003733 0 0 0; 0.0004977 0 0 0; 0.0006221 0 0 0]  x2=[0 0 0 0; 0.0001244 0 0 0; 0.0002488 0 0 0; 0.0003733 0 0 0; 0.0004977 0 0 0; 0.0006221 0 0 0]  x3=[0 0 0 0; 0.0001244 0 0 0; 0.0002488 0 0 0; 0.0003733 0 0 0; 0.0004977 0 0 0; 0.0006221 0 0 0]  x4=[0 0 0 0; 0.0001244 0 0 0; 0.0002488 0 0 0; 0.0003733 0 0 0; 0.0004977 0 0 0; 0.0006221 0 0 0]  x5=0  V1=ones(3,3)  V2=ones(3,3)  I1=ones(3,3)  I2=ones(3,3)  nHarmo=1  Measurements=None  Decoupling=off  VsMag0=0  VrMag0=0  VsAngle0=0  VrAngle0=0  IsMag0=0  IrMag0=0  IsAngle0=0  IrAngle0=0
  Distributed Parameters Line46 : powerlib/Elements/Distributed Parameters Line  Phases=3  Length=34  Frequency=50  Resistance=[0.01273 0.3864]  Inductance="[0.9337e-3  4.1264e-3]"  Capacitance=[12.74e-9 7.751e-9]  x1=[0 0 0 0; 0.0001244 0 0 0; 0.0002488 0 0 0; 0.0003733 0 0 0; 0.0004977 0 0 0; 0.0006221 0 0 0]  x2=[0 0 0 0; 0.0001244 0 0 0; 0.0002488 0 0 0; 0.0003733 0 0 0; 0.0004977 0 0 0; 0.0006221 0 0 0]  x3=[0 0 0 0; 0.0001244 0 0 0; 0.0002488 0 0 0; 0.0003733 0 0 0; 0.0004977 0 0 0; 0.0006221 0 0 0]  x4=[0 0 0 0; 0.0001244 0 0 0; 0.0002488 0 0 0; 0.0003733 0 0 0; 0.0004977 0 0 0; 0.0006221 0 0 0]  x5=0  V1=ones(3,3)  V2=ones(3,3)  I1=ones(3,3)  I2=ones(3,3)  nHarmo=1  Measurements=None  Decoupling=off  VsMag0=0  VrMag0=0  VsAngle0=0  VrAngle0=0  IsMag0=0  IrMag0=0  IsAngle0=0  IrAngle0=0
  Distributed Parameters Line47 : powerlib/Elements/Distributed Parameters Line  Phases=3  Length=18  Frequency=50  Resistance=[0.01273 0.3864]  Inductance="[0.9337e-3  4.1264e-3]"  Capacitance=[12.74e-9 7.751e-9]  x1=[0 0 0 0; 0.0001244 0 0 0; 0.0002488 0 0 0; 0.0003733 0 0 0; 0.0004977 0 0 0; 0.0006221 0 0 0]  x2=[0 0 0 0; 0.0001244 0 0 0; 0.0002488 0 0 0; 0.0003733 0 0 0; 0.0004977 0 0 0; 0.0006221 0 0 0]  x3=[0 0 0 0; 0.0001244 0 0 0; 0.0002488 0 0 0; 0.0003733 0 0 0; 0.0004977 0 0 0; 0.0006221 0 0 0]  x4=[0 0 0 0; 0.0001244 0 0 0; 0.0002488 0 0 0; 0.0003733 0 0 0; 0.0004977 0 0 0; 0.0006221 0 0 0]  x5=0  V1=ones(3,3)  V2=ones(3,3)  I1=ones(3,3)  I2=ones(3,3)  nHarmo=1  Measurements=None  Decoupling=off  VsMag0=0  VrMag0=0  VsAngle0=0  VrAngle0=0  IsMag0=0  IrMag0=0  IsAngle0=0  IrAngle0=0
  Distributed Parameters Line48 : powerlib/Elements/Distributed Parameters Line  Phases=3  Length=41  Frequency=50  Resistance=[0.01273 0.3864]  Inductance="[0.9337e-3  4.1264e-3]"  Capacitance=[12.74e-9 7.751e-9]  x1=[0 0 0 0; 0.0001244 0 0 0; 0.0002488 0 0 0; 0.0003733 0 0 0; 0.0004977 0 0 0; 0.0006221 0 0 0]  x2=[0 0 0 0; 0.0001244 0 0 0; 0.0002488 0 0 0; 0.0003733 0 0 0; 0.0004977 0 0 0; 0.0006221 0 0 0]  x3=[0 0 0 0; 0.0001244 0 0 0; 0.0002488 0 0 0; 0.0003733 0 0 0; 0.0004977 0 0 0; 0.0006221 0 0 0]  x4=[0 0 0 0; 0.0001244 0 0 0; 0.0002488 0 0 0; 0.0003733 0 0 0; 0.0004977 0 0 0; 0.0006221 0 0 0]  x5=0  V1=ones(3,3)  V2=ones(3,3)  I1=ones(3,3)  I2=ones(3,3)  nHarmo=1  Measurements=None  Decoupling=off  VsMag0=0  VrMag0=0  VsAngle0=0  VrAngle0=0  IsMag0=0  IrMag0=0  IsAngle0=0  IrAngle0=0
  Distributed Parameters Line49 : powerlib/Elements/Distributed Parameters Line  Phases=3  Length=5  Frequency=50  Resistance=[0.01273 0.3864]  Inductance="[0.9337e-3  4.1264e-3]"  Capacitance=[12.74e-9 7.751e-9]  x1=[0 0 0 0; 0.0001244 0 0 0; 0.0002488 0 0 0; 0.0003733 0 0 0; 0.0004977 0 0 0; 0.0006221 0 0 0]  x2=[0 0 0 0; 0.0001244 0 0 0; 0.0002488 0 0 0; 0.0003733 0 0 0; 0.0004977 0 0 0; 0.0006221 0 0 0]  x3=[0 0 0 0; 0.0001244 0 0 0; 0.0002488 0 0 0; 0.0003733 0 0 0; 0.0004977 0 0 0; 0.0006221 0 0 0]  x4=[0 0 0 0; 0.0001244 0 0 0; 0.0002488 0 0 0; 0.0003733 0 0 0; 0.0004977 0 0 0; 0.0006221 0 0 0]  x5=0  V1=ones(3,3)  V2=ones(3,3)  I1=ones(3,3)  I2=ones(3,3)  nHarmo=1  Measurements=None  Decoupling=off  VsMag0=0  VrMag0=0  VsAngle0=0  VrAngle0=0  IsMag0=0  IrMag0=0  IsAngle0=0  IrAngle0=0
  Distributed Parameters Line5 : powerlib/Elements/Distributed Parameters Line  Phases=3  Length=41.5  Frequency=50  Resistance=[0.01273 0.3864]  Inductance="[0.9337e-3  4.1264e-3]"  Capacitance=[12.74e-9 7.751e-9]  x1=[0 0 0 0; 0.0001244 0 0 0; 0.0002488 0 0 0; 0.0003733 0 0 0; 0.0004977 0 0 0; 0.0006221 0 0 0]  x2=[0 0 0 0; 0.0001244 0 0 0; 0.0002488 0 0 0; 0.0003733 0 0 0; 0.0004977 0 0 0; 0.0006221 0 0 0]  x3=[0 0 0 0; 0.0001244 0 0 0; 0.0002488 0 0 0; 0.0003733 0 0 0; 0.0004977 0 0 0; 0.0006221 0 0 0]  x4=[0 0 0 0; 0.0001244 0 0 0; 0.0002488 0 0 0; 0.0003733 0 0 0; 0.0004977 0 0 0; 0.0006221 0 0 0]  x5=0  V1=ones(3,3)  V2=ones(3,3)  I1=ones(3,3)  I2=ones(3,3)  nHarmo=1  Measurements=None  Decoupling=off  VsMag0=0  VrMag0=0  VsAngle0=0  VrAngle0=0  IsMag0=0  IrMag0=0  IsAngle0=0  IrAngle0=0
  Distributed Parameters Line50 : powerlib/Elements/Distributed Parameters Line  Phases=3  Length=5.5  Frequency=50  Resistance=[0.01273 0.3864]  Inductance="[0.9337e-3  4.1264e-3]"  Capacitance=[12.74e-9 7.751e-9]  x1=[0 0 0 0; 0.0001244 0 0 0; 0.0002488 0 0 0; 0.0003733 0 0 0; 0.0004977 0 0 0; 0.0006221 0 0 0]  x2=[0 0 0 0; 0.0001244 0 0 0; 0.0002488 0 0 0; 0.0003733 0 0 0; 0.0004977 0 0 0; 0.0006221 0 0 0]  x3=[0 0 0 0; 0.0001244 0 0 0; 0.0002488 0 0 0; 0.0003733 0 0 0; 0.0004977 0 0 0; 0.0006221 0 0 0]  x4=[0 0 0 0; 0.0001244 0 0 0; 0.0002488 0 0 0; 0.0003733 0 0 0; 0.0004977 0 0 0; 0.0006221 0 0 0]  x5=0  V1=ones(3,3)  V2=ones(3,3)  I1=ones(3,3)  I2=ones(3,3)  nHarmo=1  Measurements=None  Decoupling=off  VsMag0=0  VrMag0=0  VsAngle0=0  VrAngle0=0  IsMag0=0  IrMag0=0  IsAngle0=0  IrAngle0=0
  Distributed Parameters Line51 : powerlib/Elements/Distributed Parameters Line  Phases=3  Length=39.7  Frequency=50  Resistance=[0.01273 0.3864]  Inductance="[0.9337e-3  4.1264e-3]"  Capacitance=[12.74e-9 7.751e-9]  x1=[0 0 0 0; 0.0001244 0 0 0; 0.0002488 0 0 0; 0.0003733 0 0 0; 0.0004977 0 0 0; 0.0006221 0 0 0]  x2=[0 0 0 0; 0.0001244 0 0 0; 0.0002488 0 0 0; 0.0003733 0 0 0; 0.0004977 0 0 0; 0.0006221 0 0 0]  x3=[0 0 0 0; 0.0001244 0 0 0; 0.0002488 0 0 0; 0.0003733 0 0 0; 0.0004977 0 0 0; 0.0006221 0 0 0]  x4=[0 0 0 0; 0.0001244 0 0 0; 0.0002488 0 0 0; 0.0003733 0 0 0; 0.0004977 0 0 0; 0.0006221 0 0 0]  x5=0  V1=ones(3,3)  V2=ones(3,3)  I1=ones(3,3)  I2=ones(3,3)  nHarmo=1  Measurements=None  Decoupling=off  VsMag0=0  VrMag0=0  VsAngle0=0  VrAngle0=0  IsMag0=0  IrMag0=0  IsAngle0=0  IrAngle0=0
  Distributed Parameters Line52 : powerlib/Elements/Distributed Parameters Line  Phases=3  Length=55  Frequency=50  Resistance=[0.01273 0.3864]  Inductance="[0.9337e-3  4.1264e-3]"  Capacitance=[12.74e-9 7.751e-9]  x1=[0 0 0 0; 0.0001244 0 0 0; 0.0002488 0 0 0; 0.0003733 0 0 0; 0.0004977 0 0 0; 0.0006221 0 0 0]  x2=[0 0 0 0; 0.0001244 0 0 0; 0.0002488 0 0 0; 0.0003733 0 0 0; 0.0004977 0 0 0; 0.0006221 0 0 0]  x3=[0 0 0 0; 0.0001244 0 0 0; 0.0002488 0 0 0; 0.0003733 0 0 0; 0.0004977 0 0 0; 0.0006221 0 0 0]  x4=[0 0 0 0; 0.0001244 0 0 0; 0.0002488 0 0 0; 0.0003733 0 0 0; 0.0004977 0 0 0; 0.0006221 0 0 0]  x5=0  V1=ones(3,3)  V2=ones(3,3)  I1=ones(3,3)  I2=ones(3,3)  nHarmo=1  Measurements=None  Decoupling=off  VsMag0=0  VrMag0=0  VsAngle0=0  VrAngle0=0  IsMag0=0  IrMag0=0  IsAngle0=0  IrAngle0=0
  Distributed Parameters Line53 : powerlib/Elements/Distributed Parameters Line  Phases=3  Length=55  Frequency=50  Resistance=[0.01273 0.3864]  Inductance="[0.9337e-3  4.1264e-3]"  Capacitance=[12.74e-9 7.751e-9]  x1=[0 0 0 0; 0.0001244 0 0 0; 0.0002488 0 0 0; 0.0003733 0 0 0; 0.0004977 0 0 0; 0.0006221 0 0 0]  x2=[0 0 0 0; 0.0001244 0 0 0; 0.0002488 0 0 0; 0.0003733 0 0 0; 0.0004977 0 0 0; 0.0006221 0 0 0]  x3=[0 0 0 0; 0.0001244 0 0 0; 0.0002488 0 0 0; 0.0003733 0 0 0; 0.0004977 0 0 0; 0.0006221 0 0 0]  x4=[0 0 0 0; 0.0001244 0 0 0; 0.0002488 0 0 0; 0.0003733 0 0 0; 0.0004977 0 0 0; 0.0006221 0 0 0]  x5=0  V1=ones(3,3)  V2=ones(3,3)  I1=ones(3,3)  I2=ones(3,3)  nHarmo=1  Measurements=None  Decoupling=off  VsMag0=0  VrMag0=0  VsAngle0=0  VrAngle0=0  IsMag0=0  IrMag0=0  IsAngle0=0  IrAngle0=0
  Distributed Parameters Line54 : powerlib/Elements/Distributed Parameters Line  Phases=3  Length=38  Frequency=50  Resistance=[0.01273 0.3864]  Inductance="[0.9337e-3  4.1264e-3]"  Capacitance=[12.74e-9 7.751e-9]  x1=[0 0 0 0; 0.0001244 0 0 0; 0.0002488 0 0 0; 0.0003733 0 0 0; 0.0004977 0 0 0; 0.0006221 0 0 0]  x2=[0 0 0 0; 0.0001244 0 0 0; 0.0002488 0 0 0; 0.0003733 0 0 0; 0.0004977 0 0 0; 0.0006221 0 0 0]  x3=[0 0 0 0; 0.0001244 0 0 0; 0.0002488 0 0 0; 0.0003733 0 0 0; 0.0004977 0 0 0; 0.0006221 0 0 0]  x4=[0 0 0 0; 0.0001244 0 0 0; 0.0002488 0 0 0; 0.0003733 0 0 0; 0.0004977 0 0 0; 0.0006221 0 0 0]  x5=0  V1=ones(3,3)  V2=ones(3,3)  I1=ones(3,3)  I2=ones(3,3)  nHarmo=1  Measurements=None  Decoupling=off  VsMag0=0  VrMag0=0  VsAngle0=0  VrAngle0=0  IsMag0=0  IrMag0=0  IsAngle0=0  IrAngle0=0
  Distributed Parameters Line55 : powerlib/Elements/Distributed Parameters Line  Phases=3  Length=38  Frequency=50  Resistance=[0.01273 0.3864]  Inductance="[0.9337e-3  4.1264e-3]"  Capacitance=[12.74e-9 7.751e-9]  x1=[0 0 0 0; 0.0001244 0 0 0; 0.0002488 0 0 0; 0.0003733 0 0 0; 0.0004977 0 0 0; 0.0006221 0 0 0]  x2=[0 0 0 0; 0.0001244 0 0 0; 0.0002488 0 0 0; 0.0003733 0 0 0; 0.0004977 0 0 0; 0.0006221 0 0 0]  x3=[0 0 0 0; 0.0001244 0 0 0; 0.0002488 0 0 0; 0.0003733 0 0 0; 0.0004977 0 0 0; 0.0006221 0 0 0]  x4=[0 0 0 0; 0.0001244 0 0 0; 0.0002488 0 0 0; 0.0003733 0 0 0; 0.0004977 0 0 0; 0.0006221 0 0 0]  x5=0  V1=ones(3,3)  V2=ones(3,3)  I1=ones(3,3)  I2=ones(3,3)  nHarmo=1  Measurements=None  Decoupling=off  VsMag0=0  VrMag0=0  VsAngle0=0  VrAngle0=0  IsMag0=0  IrMag0=0  IsAngle0=0  IrAngle0=0
  Distributed Parameters Line56 : powerlib/Elements/Distributed Parameters Line  Phases=3  Length=72.5  Frequency=50  Resistance=[0.01273 0.3864]  Inductance="[0.9337e-3  4.1264e-3]"  Capacitance=[12.74e-9 7.751e-9]  x1=[0 0 0 0; 0.0001244 0 0 0; 0.0002488 0 0 0; 0.0003733 0 0 0; 0.0004977 0 0 0; 0.0006221 0 0 0]  x2=[0 0 0 0; 0.0001244 0 0 0; 0.0002488 0 0 0; 0.0003733 0 0 0; 0.0004977 0 0 0; 0.0006221 0 0 0]  x3=[0 0 0 0; 0.0001244 0 0 0; 0.0002488 0 0 0; 0.0003733 0 0 0; 0.0004977 0 0 0; 0.0006221 0 0 0]  x4=[0 0 0 0; 0.0001244 0 0 0; 0.0002488 0 0 0; 0.0003733 0 0 0; 0.0004977 0 0 0; 0.0006221 0 0 0]  x5=0  V1=ones(3,3)  V2=ones(3,3)  I1=ones(3,3)  I2=ones(3,3)  nHarmo=1  Measurements=None  Decoupling=off  VsMag0=0  VrMag0=0  VsAngle0=0  VrAngle0=0  IsMag0=0  IrMag0=0  IsAngle0=0  IrAngle0=0
  Distributed Parameters Line57 : powerlib/Elements/Distributed Parameters Line  Phases=3  Length=72.5  Frequency=50  Resistance=[0.01273 0.3864]  Inductance="[0.9337e-3  4.1264e-3]"  Capacitance=[12.74e-9 7.751e-9]  x1=[0 0 0 0; 0.0001244 0 0 0; 0.0002488 0 0 0; 0.0003733 0 0 0; 0.0004977 0 0 0; 0.0006221 0 0 0]  x2=[0 0 0 0; 0.0001244 0 0 0; 0.0002488 0 0 0; 0.0003733 0 0 0; 0.0004977 0 0 0; 0.0006221 0 0 0]  x3=[0 0 0 0; 0.0001244 0 0 0; 0.0002488 0 0 0; 0.0003733 0 0 0; 0.0004977 0 0 0; 0.0006221 0 0 0]  x4=[0 0 0 0; 0.0001244 0 0 0; 0.0002488 0 0 0; 0.0003733 0 0 0; 0.0004977 0 0 0; 0.0006221 0 0 0]  x5=0  V1=ones(3,3)  V2=ones(3,3)  I1=ones(3,3)  I2=ones(3,3)  nHarmo=1  Measurements=None  Decoupling=off  VsMag0=0  VrMag0=0  VsAngle0=0  VrAngle0=0  IsMag0=0  IrMag0=0  IsAngle0=0  IrAngle0=0
  Distributed Parameters Line58 : powerlib/Elements/Distributed Parameters Line  Phases=3  Length=106  Frequency=50  Resistance=[0.01273 0.3864]  Inductance="[0.9337e-3  4.1264e-3]"  Capacitance=[12.74e-9 7.751e-9]  x1=[0 0 0 0; 0.0001244 0 0 0; 0.0002488 0 0 0; 0.0003733 0 0 0; 0.0004977 0 0 0; 0.0006221 0 0 0]  x2=[0 0 0 0; 0.0001244 0 0 0; 0.0002488 0 0 0; 0.0003733 0 0 0; 0.0004977 0 0 0; 0.0006221 0 0 0]  x3=[0 0 0 0; 0.0001244 0 0 0; 0.0002488 0 0 0; 0.0003733 0 0 0; 0.0004977 0 0 0; 0.0006221 0 0 0]  x4=[0 0 0 0; 0.0001244 0 0 0; 0.0002488 0 0 0; 0.0003733 0 0 0; 0.0004977 0 0 0; 0.0006221 0 0 0]  x5=0  V1=ones(3,3)  V2=ones(3,3)  I1=ones(3,3)  I2=ones(3,3)  nHarmo=1  Measurements=None  Decoupling=off  VsMag0=0  VrMag0=0  VsAngle0=0  VrAngle0=0  IsMag0=0  IrMag0=0  IsAngle0=0  IrAngle0=0
  Distributed Parameters Line59 : powerlib/Elements/Distributed Parameters Line  Phases=3  Length=106  Frequency=50  Resistance=[0.01273 0.3864]  Inductance="[0.9337e-3  4.1264e-3]"  Capacitance=[12.74e-9 7.751e-9]  x1=[0 0 0 0; 0.0001244 0 0 0; 0.0002488 0 0 0; 0.0003733 0 0 0; 0.0004977 0 0 0; 0.0006221 0 0 0]  x2=[0 0 0 0; 0.0001244 0 0 0; 0.0002488 0 0 0; 0.0003733 0 0 0; 0.0004977 0 0 0; 0.0006221 0 0 0]  x3=[0 0 0 0; 0.0001244 0 0 0; 0.0002488 0 0 0; 0.0003733 0 0 0; 0.0004977 0 0 0; 0.0006221 0 0 0]  x4=[0 0 0 0; 0.0001244 0 0 0; 0.0002488 0 0 0; 0.0003733 0 0 0; 0.0004977 0 0 0; 0.0006221 0 0 0]  x5=0  V1=ones(3,3)  V2=ones(3,3)  I1=ones(3,3)  I2=ones(3,3)  nHarmo=1  Measurements=None  Decoupling=off  VsMag0=0  VrMag0=0  VsAngle0=0  VrAngle0=0  IsMag0=0  IrMag0=0  IsAngle0=0  IrAngle0=0
  Distributed Parameters Line6 : powerlib/Elements/Distributed Parameters Line  Phases=3  Length=41.5  Frequency=50  Resistance=[0.01273 0.3864]  Inductance="[0.9337e-3  4.1264e-3]"  Capacitance=[12.74e-9 7.751e-9]  x1=[0 0 0 0; 0.0001244 0 0 0; 0.0002488 0 0 0; 0.0003733 0 0 0; 0.0004977 0 0 0; 0.0006221 0 0 0]  x2=[0 0 0 0; 0.0001244 0 0 0; 0.0002488 0 0 0; 0.0003733 0 0 0; 0.0004977 0 0 0; 0.0006221 0 0 0]  x3=[0 0 0 0; 0.0001244 0 0 0; 0.0002488 0 0 0; 0.0003733 0 0 0; 0.0004977 0 0 0; 0.0006221 0 0 0]  x4=[0 0 0 0; 0.0001244 0 0 0; 0.0002488 0 0 0; 0.0003733 0 0 0; 0.0004977 0 0 0; 0.0006221 0 0 0]  x5=0  V1=ones(3,3)  V2=ones(3,3)  I1=ones(3,3)  I2=ones(3,3)  nHarmo=1  Measurements=None  Decoupling=off  VsMag0=0  VrMag0=0  VsAngle0=0  VrAngle0=0  IsMag0=0  IrMag0=0  IsAngle0=0  IrAngle0=0
  Ground : powerlib/Elements/Ground  LConnTagsString=a
  Ground1 : powerlib/Elements/Ground  LConnTagsString=a
  Ishwardi : powerlib/Measurements/Three-Phase V-I Measurement  VoltageMeasurement=no  SetLabelV=off  LabelV=Vabc  Vpu=off  VpuLL=off  CurrentMeasurement=no  SetLabelI=off  LabelI=Iabc  Ipu=off  Pbase=100e6  Vbase=500e3  OutputType=Complex  PhasorSimulation=off  PSBequivalent=0
  Ishwardi PP : powerlib/Measurements/Three-Phase V-I Measurement  VoltageMeasurement=no  SetLabelV=off  LabelV=Vabc  Vpu=off  VpuLL=off  CurrentMeasurement=no  SetLabelI=off  LabelI=Iabc  Ipu=off  Pbase=100e6  Vbase=500e3  OutputType=Complex  PhasorSimulation=off  PSBequivalent=0
  Jaldhaka : powerlib/Measurements/Three-Phase V-I Measurement  VoltageMeasurement=no  SetLabelV=off  LabelV=Vabc  Vpu=off  VpuLL=off  CurrentMeasurement=no  SetLabelI=off  LabelI=Iabc  Ipu=off  Pbase=100e6  Vbase=500e3  OutputType=Complex  PhasorSimulation=off  PSBequivalent=0
  Joypurhat : powerlib/Measurements/Three-Phase V-I Measurement  VoltageMeasurement=no  SetLabelV=off  LabelV=Vabc  Vpu=off  VpuLL=off  CurrentMeasurement=no  SetLabelI=off  LabelI=Iabc  Ipu=off  Pbase=100e6  Vbase=500e3  OutputType=Complex  PhasorSimulation=off  PSBequivalent=0
  Kurigram : powerlib/Measurements/Three-Phase V-I Measurement  VoltageMeasurement=no  SetLabelV=off  LabelV=Vabc  Vpu=off  VpuLL=off  CurrentMeasurement=no  SetLabelI=off  LabelI=Iabc  Ipu=off  Pbase=100e6  Vbase=500e3  OutputType=Complex  PhasorSimulation=off  PSBequivalent=0
  Lalmonirhat : powerlib/Measurements/Three-Phase V-I Measurement  VoltageMeasurement=no  SetLabelV=off  LabelV=Vabc  Vpu=off  VpuLL=off  CurrentMeasurement=no  SetLabelI=off  LabelI=Iabc  Ipu=off  Pbase=100e6  Vbase=500e3  OutputType=Complex  PhasorSimulation=off  PSBequivalent=0
  Mahastangarh : powerlib/Measurements/Three-Phase V-I Measurement  VoltageMeasurement=no  SetLabelV=off  LabelV=Vabc  Vpu=off  VpuLL=off  CurrentMeasurement=no  SetLabelI=off  LabelI=Iabc  Ipu=off  Pbase=100e6  Vbase=500e3  OutputType=Complex  PhasorSimulation=off  PSBequivalent=0
  Naogaon : powerlib/Measurements/Three-Phase V-I Measurement  VoltageMeasurement=no  SetLabelV=off  LabelV=Vabc  Vpu=off  VpuLL=off  CurrentMeasurement=no  SetLabelI=off  LabelI=Iabc  Ipu=off  Pbase=100e6  Vbase=500e3  OutputType=Complex  PhasorSimulation=off  PSBequivalent=0
  Natore : powerlib/Measurements/Three-Phase V-I Measurement  VoltageMeasurement=no  SetLabelV=off  LabelV=Vabc  Vpu=off  VpuLL=off  CurrentMeasurement=no  SetLabelI=off  LabelI=Iabc  Ipu=off  Pbase=100e6  Vbase=500e3  OutputType=Complex  PhasorSimulation=off  PSBequivalent=0
  Niyamotpur : powerlib/Measurements/Three-Phase V-I Measurement  VoltageMeasurement=no  SetLabelV=off  LabelV=Vabc  Vpu=off  VpuLL=off  CurrentMeasurement=no  SetLabelI=off  LabelI=Iabc  Ipu=off  Pbase=100e6  Vbase=500e3  OutputType=Complex  PhasorSimulation=off  PSBequivalent=0
  Pabna : powerlib/Measurements/Three-Phase V-I Measurement  VoltageMeasurement=no  SetLabelV=off  LabelV=Vabc  Vpu=off  VpuLL=off  CurrentMeasurement=no  SetLabelI=off  LabelI=Iabc  Ipu=off  Pbase=100e6  Vbase=500e3  OutputType=Complex  PhasorSimulation=off  PSBequivalent=0
  Palashbari : powerlib/Measurements/Three-Phase V-I Measurement  VoltageMeasurement=phase-to-ground  SetLabelV=off  LabelV=Vabc  Vpu=off  VpuLL=off  CurrentMeasurement=yes  SetLabelI=off  LabelI=Iabc  Ipu=off  Pbase=100e6  Vbase=500e3  OutputType=Complex  PhasorSimulation=off  PSBequivalent=0
  Panchagarh : powerlib/Measurements/Three-Phase V-I Measurement  VoltageMeasurement=no  SetLabelV=off  LabelV=Vabc  Vpu=off  VpuLL=off  CurrentMeasurement=no  SetLabelI=off  LabelI=Iabc  Ipu=off  Pbase=100e6  Vbase=500e3  OutputType=Complex  PhasorSimulation=off  PSBequivalent=0
  Purba Sadipur : powerlib/Measurements/Three-Phase V-I Measurement  VoltageMeasurement=no  SetLabelV=off  LabelV=Vabc  Vpu=off  VpuLL=off  CurrentMeasurement=no  SetLabelI=off  LabelI=Iabc  Ipu=off  Pbase=100e6  Vbase=500e3  OutputType=Complex  PhasorSimulation=off  PSBequivalent=0
  Rajshahi : powerlib/Measurements/Three-Phase V-I Measurement  VoltageMeasurement=no  SetLabelV=off  LabelV=Vabc  Vpu=off  VpuLL=off  CurrentMeasurement=no  SetLabelI=off  LabelI=Iabc  Ipu=off  Pbase=100e6  Vbase=500e3  OutputType=Complex  PhasorSimulation=off  PSBequivalent=0
  Rajshahi (N) : powerlib/Measurements/Three-Phase V-I Measurement  VoltageMeasurement=no  SetLabelV=off  LabelV=Vabc  Vpu=off  VpuLL=off  CurrentMeasurement=no  SetLabelI=off  LabelI=Iabc  Ipu=off  Pbase=100e6  Vbase=500e3  OutputType=Complex  PhasorSimulation=off  PSBequivalent=0
  Rangpur : powerlib/Measurements/Three-Phase V-I Measurement  VoltageMeasurement=no  SetLabelV=off  LabelV=Vabc  Vpu=off  VpuLL=off  CurrentMeasurement=no  SetLabelI=off  LabelI=Iabc  Ipu=off  Pbase=100e6  Vbase=500e3  OutputType=Complex  PhasorSimulation=off  PSBequivalent=0
  Rooppur : powerlib/Measurements/Three-Phase V-I Measurement  VoltageMeasurement=no  SetLabelV=off  LabelV=Vabc  Vpu=off  VpuLL=off  CurrentMeasurement=no  SetLabelI=off  LabelI=Iabc  Ipu=off  Pbase=100e6  Vbase=500e3  OutputType=Complex  PhasorSimulation=off  PSBequivalent=0
  Saidpur : powerlib/Measurements/Three-Phase V-I Measurement  VoltageMeasurement=no  SetLabelV=off  LabelV=Vabc  Vpu=off  VpuLL=off  CurrentMeasurement=no  SetLabelI=off  LabelI=Iabc  Ipu=off  Pbase=100e6  Vbase=500e3  OutputType=Complex  PhasorSimulation=off  PSBequivalent=0
  Scope : Scope  NumInputPorts=3
  Scope1 : Scope  NumInputPorts=3
  Scope2 : Scope
  Scope3 : Scope
  Series RLC Branch : powerlib/Elements/Series RLC Branch  LConnTagsString=__new0  RConnTagsString=__new0  BranchType=C  Resistance=1  Inductance=1e-3  SetiL0=off  InitialCurrent=0  Capacitance=8.22e-6  Setx0=off  InitialVoltage=0  Measurements=None
  Series RLC Branch1 : powerlib/Elements/Series RLC Branch  LConnTagsString=__new0  RConnTagsString=__new0  BranchType=C  Resistance=1  Inductance=1e-3  SetiL0=off  InitialCurrent=0  Capacitance=8.22e-6  Setx0=off  InitialVoltage=0  Measurements=None
  Series RLC Branch2 : powerlib/Elements/Series RLC Branch  LConnTagsString=__new0  RConnTagsString=__new0  BranchType=C  Resistance=1  Inductance=1e-3  SetiL0=off  InitialCurrent=0  Capacitance=8.22e-6  Setx0=off  InitialVoltage=0  Measurements=None
  Shahjadpur : powerlib/Measurements/Three-Phase V-I Measurement  VoltageMeasurement=no  SetLabelV=off  LabelV=Vabc  Vpu=off  VpuLL=off  CurrentMeasurement=no  SetLabelI=off  LabelI=Iabc  Ipu=off  Pbase=100e6  Vbase=500e3  OutputType=Complex  PhasorSimulation=off  PSBequivalent=0
  Sherpur (B) : powerlib/Measurements/Three-Phase V-I Measurement  VoltageMeasurement=no  SetLabelV=off  LabelV=Vabc  Vpu=off  VpuLL=off  CurrentMeasurement=no  SetLabelI=off  LabelI=Iabc  Ipu=off  Pbase=100e6  Vbase=500e3  OutputType=Complex  PhasorSimulation=off  PSBequivalent=0
  Sirajganj : powerlib/Measurements/Three-Phase V-I Measurement  VoltageMeasurement=no  SetLabelV=off  LabelV=Vabc  Vpu=off  VpuLL=off  CurrentMeasurement=no  SetLabelI=off  LabelI=Iabc  Ipu=off  Pbase=100e6  Vbase=500e3  OutputType=Complex  PhasorSimulation=off  PSBequivalent=0
  Sirajganj SW PP : powerlib/Measurements/Three-Phase V-I Measurement  VoltageMeasurement=no  SetLabelV=off  LabelV=Vabc  Vpu=off  VpuLL=off  CurrentMeasurement=no  SetLabelI=off  LabelI=Iabc  Ipu=off  Pbase=100e6  Vbase=500e3  OutputType=Complex  PhasorSimulation=off  PSBequivalent=0
  Subsystem : Subsystem
  Subsystem1 : Subsystem
  Subsystem10 : Subsystem
  Subsystem11 : Subsystem
  Subsystem12 : Subsystem
  Subsystem13 : Subsystem
  Subsystem14 : Subsystem
  Subsystem15 : Subsystem
  Subsystem16 : Subsystem
  Subsystem17 : Subsystem
  Subsystem18 : Subsystem
  Subsystem19 : Subsystem
  Subsystem2 : Subsystem
  Subsystem20 : Subsystem
  Subsystem21 : Subsystem
  Subsystem22 : Subsystem
  Subsystem23 : Subsystem
  Subsystem24 : Subsystem
  Subsystem25 : Subsystem
  Subsystem26 : Subsystem
  Subsystem3 : Subsystem
  Subsystem4 : Subsystem
  Subsystem5 : Subsystem
  Subsystem6 : Subsystem
  Subsystem7 : Subsystem
  Subsystem8 : Subsystem
  Subsystem9 : Subsystem
  Thakurgaon : powerlib/Measurements/Three-Phase V-I Measurement  VoltageMeasurement=no  SetLabelV=off  LabelV=Vabc  Vpu=off  VpuLL=off  CurrentMeasurement=no  SetLabelI=off  LabelI=Iabc  Ipu=off  Pbase=100e6  Vbase=500e3  OutputType=Complex  PhasorSimulation=off  PSBequivalent=0
  Three-Phase Transformer (Two Windings){86..87,89..90,92,94..96} (8 alike) : powerlib/Elements/Three-Phase Transformer (Two Windings)  Winding1Connection=Delta (D1)  Winding2Connection=Yg  CoreType=Three single-phase transformers  SetSaturation=off  Hysteresis=off  DataFile='hysteresis'  SetInitialFlux=off  Measurements=None  UNITS=pu  NominalPower=[ 225e6 , 50 ]  Winding1=[ 230e3 , 0.002 , 0.08 ]  Winding2=[132e3 , 0.002 , 0.08 ]  Rm=500  Lm=500  L0=0.5  Saturation=[ 0,0 ; 0.0024,1.2 ; 1.0,1.52 ]  InitialFluxes=[ 0.8 , -0.8 , 0.7 ]  BreakLoop=off  DiscreteSolver=Trapezoidal iterative  DataType=off  TransfoNumber=1
  Three-Phase Transformer (Two Windings)88 : powerlib/Elements/Three-Phase Transformer (Two Windings)  Winding1Connection=Delta (D1)  Winding2Connection=Yg  CoreType=Three single-phase transformers  SetSaturation=off  Hysteresis=off  DataFile='hysteresis'  SetInitialFlux=off  Measurements=None  UNITS=pu  NominalPower=[ 300e6 , 50 ]  Winding1=[ 230e3 , 0.002 , 0.08 ]  Winding2=[132e3 , 0.002 , 0.08 ]  Rm=500  Lm=500  L0=0.5  Saturation=[ 0,0 ; 0.0024,1.2 ; 1.0,1.52 ]  InitialFluxes=[ 0.8 , -0.8 , 0.7 ]  BreakLoop=off  DiscreteSolver=Trapezoidal iterative  DataType=off  TransfoNumber=1
  Three-Phase Transformer (Two Windings)91 : powerlib/Elements/Three-Phase Transformer (Two Windings)  Winding1Connection=Delta (D1)  Winding2Connection=Yg  CoreType=Three single-phase transformers  SetSaturation=off  Hysteresis=off  DataFile='hysteresis'  SetInitialFlux=off  Measurements=None  UNITS=pu  NominalPower=[ 300e6 , 50 ]  Winding1=[ 230e3 , 0.002 , 0.08 ]  Winding2=[132e3 , 0.002 , 0.08 ]  Rm=500  Lm=500  L0=0.5  Saturation=[ 0,0 ; 0.0024,1.2 ; 1.0,1.52 ]  InitialFluxes=[ 0.8 , -0.8 , 0.7 ]  BreakLoop=off  DiscreteSolver=Trapezoidal iterative  DataType=off  TransfoNumber=1
  Three-Phase Transformer (Two Windings)93 : powerlib/Elements/Three-Phase Transformer (Two Windings)  Winding1Connection=Delta (D1)  Winding2Connection=Yg  CoreType=Three single-phase transformers  SetSaturation=off  Hysteresis=off  DataFile='hysteresis'  SetInitialFlux=off  Measurements=None  UNITS=pu  NominalPower=[ 300e6 , 50 ]  Winding1=[ 230e3 , 0.002 , 0.08 ]  Winding2=[132e3 , 0.002 , 0.08 ]  Rm=500  Lm=500  L0=0.5  Saturation=[ 0,0 ; 0.0024,1.2 ; 1.0,1.52 ]  InitialFluxes=[ 0.8 , -0.8 , 0.7 ]  BreakLoop=off  DiscreteSolver=Trapezoidal iterative  DataType=off  TransfoNumber=1
  Three-Phase Fault : powerlib/Elements/Three-Phase Fault  InitialStates=0  FaultA=on  FaultB=on  FaultC=off  GroundFault=off  SwitchTimes="[1/100  3/100]"  External=off  SwitchStatus=NaN  FaultResistance=0.001  GroundResistance=0.01  SnubberResistance=1e6  SnubberCapacitance=inf  Measurements=None
  Three-Phase Source : powerlib/Electrical Sources/Three-Phase Source  InternalConnection=Yg  VoltagePhases=off  Voltage=132e3  PhaseAngle=0  Voltage_phases=[25e3 25e3 25e3]/sqrt(3)  PhaseAngles_phases=[0 -120 +120]  Frequency=50  NonIdealSource=on  SpecifyImpedance=off  Resistance=0.8929  Inductance=16.58e-3  ShortCircuitLevel=2e6  BaseVoltage=132e3  XRratio=7  BusType=PV  Pref=20e6  Qref=0  Prefabc=[10e3, 10e3, 10e3]  Qrefabc=[0, 0, 0]  Qmin=-100  Qmax=100
  Three-Phase Source1 : powerlib/Electrical Sources/Three-Phase Source  InternalConnection=Yg  VoltagePhases=off  Voltage=132e3  PhaseAngle=0  Voltage_phases=[25e3 25e3 25e3]/sqrt(3)  PhaseAngles_phases=[0 -120 +120]  Frequency=50  NonIdealSource=on  SpecifyImpedance=off  Resistance=0.8929  Inductance=16.58e-3  ShortCircuitLevel=100e6  BaseVoltage=132e3  XRratio=7  BusType=PV  Pref=20e6  Qref=0  Prefabc=[10e3, 10e3, 10e3]  Qrefabc=[0, 0, 0]  Qmin=-inf  Qmax=inf
  Three-Phase Source10 : powerlib/Electrical Sources/Three-Phase Source  InternalConnection=Yg  VoltagePhases=off  Voltage=132e3  PhaseAngle=0  Voltage_phases=[25e3 25e3 25e3]/sqrt(3)  PhaseAngles_phases=[0 -120 +120]  Frequency=50  NonIdealSource=on  SpecifyImpedance=off  Resistance=0.8929  Inductance=16.58e-3  ShortCircuitLevel=50e6  BaseVoltage=132e3  XRratio=7  BusType=PV  Pref=100e6  Qref=0  Prefabc=[10e3, 10e3, 10e3]  Qrefabc=[0, 0, 0]  Qmin=-inf  Qmax=inf
  Three-Phase Source11 : powerlib/Electrical Sources/Three-Phase Source  InternalConnection=Yg  VoltagePhases=off  Voltage=132e3  PhaseAngle=0  Voltage_phases=[25e3 25e3 25e3]/sqrt(3)  PhaseAngles_phases=[0 -120 +120]  Frequency=50  NonIdealSource=on  SpecifyImpedance=off  Resistance=0.8929  Inductance=16.58e-3  ShortCircuitLevel=50e6  BaseVoltage=132e3  XRratio=7  BusType=PV  Pref=70e6  Qref=0  Prefabc=[10e3, 10e3, 10e3]  Qrefabc=[0, 0, 0]  Qmin=-inf  Qmax=inf
  Three-Phase Source12 : powerlib/Electrical Sources/Three-Phase Source  InternalConnection=Yg  VoltagePhases=off  Voltage=132e3  PhaseAngle=0  Voltage_phases=[25e3 25e3 25e3]/sqrt(3)  PhaseAngles_phases=[0 -120 +120]  Frequency=50  NonIdealSource=on  SpecifyImpedance=off  Resistance=0.8929  Inductance=16.58e-3  ShortCircuitLevel=50e6  BaseVoltage=132e3  XRratio=7  BusType=PV  Pref=52e6  Qref=0  Prefabc=[10e3, 10e3, 10e3]  Qrefabc=[0, 0, 0]  Qmin=-inf  Qmax=inf
  Three-Phase Source13 : powerlib/Electrical Sources/Three-Phase Source  InternalConnection=Yg  VoltagePhases=off  Voltage=132e3  PhaseAngle=0  Voltage_phases=[25e3 25e3 25e3]/sqrt(3)  PhaseAngles_phases=[0 -120 +120]  Frequency=50  NonIdealSource=on  SpecifyImpedance=off  Resistance=0.8929  Inductance=16.58e-3  ShortCircuitLevel=50e6  BaseVoltage=132e3  XRratio=7  BusType=PV  Pref=71e6  Qref=0  Prefabc=[10e3, 10e3, 10e3]  Qrefabc=[0, 0, 0]  Qmin=-inf  Qmax=inf
  Three-Phase Source14 : powerlib/Electrical Sources/Three-Phase Source  InternalConnection=Yg  VoltagePhases=off  Voltage=132e3  PhaseAngle=0  Voltage_phases=[25e3 25e3 25e3]/sqrt(3)  PhaseAngles_phases=[0 -120 +120]  Frequency=50  NonIdealSource=on  SpecifyImpedance=off  Resistance=0.8929  Inductance=16.58e-3  ShortCircuitLevel=50e6  BaseVoltage=132e3  XRratio=7  BusType=PV  Pref=100e6  Qref=0  Prefabc=[10e3, 10e3, 10e3]  Qrefabc=[0, 0, 0]  Qmin=-inf  Qmax=inf
  Three-Phase Source15 : powerlib/Electrical Sources/Three-Phase Source  InternalConnection=Yg  VoltagePhases=off  Voltage=132e3  PhaseAngle=0  Voltage_phases=[25e3 25e3 25e3]/sqrt(3)  PhaseAngles_phases=[0 -120 +120]  Frequency=50  NonIdealSource=on  SpecifyImpedance=off  Resistance=0.8929  Inductance=16.58e-3  ShortCircuitLevel=50e6  BaseVoltage=132e3  XRratio=7  BusType=PV  Pref=33e6  Qref=0  Prefabc=[10e3, 10e3, 10e3]  Qrefabc=[0, 0, 0]  Qmin=-inf  Qmax=inf
  Three-Phase Source16 : powerlib/Electrical Sources/Three-Phase Source  InternalConnection=Yg  VoltagePhases=off  Voltage=132e3  PhaseAngle=0  Voltage_phases=[25e3 25e3 25e3]/sqrt(3)  PhaseAngles_phases=[0 -120 +120]  Frequency=50  NonIdealSource=on  SpecifyImpedance=off  Resistance=0.8929  Inductance=16.58e-3  ShortCircuitLevel=50e6  BaseVoltage=132e3  XRratio=7  BusType=PV  Pref=16e6  Qref=0  Prefabc=[10e3, 10e3, 10e3]  Qrefabc=[0, 0, 0]  Qmin=-inf  Qmax=inf
  Three-Phase Source17 : powerlib/Electrical Sources/Three-Phase Source  InternalConnection=Yg  VoltagePhases=off  Voltage=132e3  PhaseAngle=0  Voltage_phases=[25e3 25e3 25e3]/sqrt(3)  PhaseAngles_phases=[0 -120 +120]  Frequency=50  NonIdealSource=on  SpecifyImpedance=off  Resistance=0.8929  Inductance=16.58e-3  ShortCircuitLevel=50e6  BaseVoltage=132e3  XRratio=7  BusType=PV  Pref=16e6  Qref=0  Prefabc=[10e3, 10e3, 10e3]  Qrefabc=[0, 0, 0]  Qmin=-inf  Qmax=inf
  Three-Phase Source18 : powerlib/Electrical Sources/Three-Phase Source  InternalConnection=Yg  VoltagePhases=off  Voltage=132e3  PhaseAngle=0  Voltage_phases=[25e3 25e3 25e3]/sqrt(3)  PhaseAngles_phases=[0 -120 +120]  Frequency=50  NonIdealSource=on  SpecifyImpedance=off  Resistance=0.8929  Inductance=16.58e-3  ShortCircuitLevel=50e6  BaseVoltage=132e3  XRratio=7  BusType=PV  Pref=16e6  Qref=0  Prefabc=[10e3, 10e3, 10e3]  Qrefabc=[0, 0, 0]  Qmin=-inf  Qmax=inf
  Three-Phase Source19 : powerlib/Electrical Sources/Three-Phase Source  InternalConnection=Yg  VoltagePhases=off  Voltage=132e3  PhaseAngle=0  Voltage_phases=[25e3 25e3 25e3]/sqrt(3)  PhaseAngles_phases=[0 -120 +120]  Frequency=50  NonIdealSource=on  SpecifyImpedance=off  Resistance=0.8929  Inductance=16.58e-3  ShortCircuitLevel=50e6  BaseVoltage=132e3  XRratio=7  BusType=PV  Pref=160e6  Qref=0  Prefabc=[10e3, 10e3, 10e3]  Qrefabc=[0, 0, 0]  Qmin=-inf  Qmax=inf
  Three-Phase Source2 : powerlib/Electrical Sources/Three-Phase Source  InternalConnection=Yn  VoltagePhases=off  Voltage=132e3  PhaseAngle=0  Voltage_phases=[25e3 25e3 25e3]/sqrt(3)  PhaseAngles_phases=[0 -120 +120]  Frequency=50  NonIdealSource=on  SpecifyImpedance=off  Resistance=0.8929  Inductance=16.58e-3  ShortCircuitLevel=100e6  BaseVoltage=132e3  XRratio=7  BusType=PV  Pref=113e6  Qref=0  Prefabc=[10e3, 10e3, 10e3]  Qrefabc=[0, 0, 0]  Qmin=-inf  Qmax=inf
  Three-Phase Source20 : powerlib/Electrical Sources/Three-Phase Source  InternalConnection=Yg  VoltagePhases=off  Voltage=230e3  PhaseAngle=0  Voltage_phases=[25e3 25e3 25e3]/sqrt(3)  PhaseAngles_phases=[0 -120 +120]  Frequency=50  NonIdealSource=on  SpecifyImpedance=off  Resistance=0.8929  Inductance=16.58e-3  ShortCircuitLevel=50e6  BaseVoltage=230e3  XRratio=7  BusType=PV  Pref=200e6  Qref=0  Prefabc=[10e3, 10e3, 10e3]  Qrefabc=[0, 0, 0]  Qmin=-inf  Qmax=inf
  Three-Phase Source21 : powerlib/Electrical Sources/Three-Phase Source  InternalConnection=Yg  VoltagePhases=off  Voltage=230e3  PhaseAngle=0  Voltage_phases=[25e3 25e3 25e3]/sqrt(3)  PhaseAngles_phases=[0 -120 +120]  Frequency=50  NonIdealSource=on  SpecifyImpedance=off  Resistance=0.8929  Inductance=16.58e-3  ShortCircuitLevel=50e6  BaseVoltage=230e3  XRratio=7  BusType=PV  Pref=225e6  Qref=0  Prefabc=[10e3, 10e3, 10e3]  Qrefabc=[0, 0, 0]  Qmin=-inf  Qmax=inf
  Three-Phase Source22 : powerlib/Electrical Sources/Three-Phase Source  InternalConnection=Yg  VoltagePhases=off  Voltage=230e3  PhaseAngle=0  Voltage_phases=[25e3 25e3 25e3]/sqrt(3)  PhaseAngles_phases=[0 -120 +120]  Frequency=50  NonIdealSource=on  SpecifyImpedance=off  Resistance=0.8929  Inductance=16.58e-3  ShortCircuitLevel=50e6  BaseVoltage=230e3  XRratio=7  BusType=PV  Pref=225e6  Qref=0  Prefabc=[10e3, 10e3, 10e3]  Qrefabc=[0, 0, 0]  Qmin=-inf  Qmax=inf
  Three-Phase Source23 : powerlib/Electrical Sources/Three-Phase Source  InternalConnection=Yg  VoltagePhases=off  Voltage=230e3  PhaseAngle=0  Voltage_phases=[25e3 25e3 25e3]/sqrt(3)  PhaseAngles_phases=[0 -120 +120]  Frequency=50  NonIdealSource=on  SpecifyImpedance=off  Resistance=0.8929  Inductance=16.58e-3  ShortCircuitLevel=50e6  BaseVoltage=230e3  XRratio=7  BusType=PV  Pref=225e6  Qref=0  Prefabc=[10e3, 10e3, 10e3]  Qrefabc=[0, 0, 0]  Qmin=-inf  Qmax=inf
  Three-Phase Source24 : powerlib/Electrical Sources/Three-Phase Source  InternalConnection=Yg  VoltagePhases=off  Voltage=230e3  PhaseAngle=0  Voltage_phases=[25e3 25e3 25e3]/sqrt(3)  PhaseAngles_phases=[0 -120 +120]  Frequency=50  NonIdealSource=on  SpecifyImpedance=off  Resistance=0.8929  Inductance=16.58e-3  ShortCircuitLevel=50e6  BaseVoltage=230e3  XRratio=7  BusType=PV  Pref=414e6  Qref=0  Prefabc=[10e3, 10e3, 10e3]  Qrefabc=[0, 0, 0]  Qmin=-inf  Qmax=inf
  Three-Phase Source25 : powerlib/Electrical Sources/Three-Phase Source  InternalConnection=Yg  VoltagePhases=off  Voltage=132e3  PhaseAngle=0  Voltage_phases=[25e3 25e3 25e3]/sqrt(3)  PhaseAngles_phases=[0 -120 +120]  Frequency=50  NonIdealSource=on  SpecifyImpedance=off  Resistance=0.8929  Inductance=16.58e-3  ShortCircuitLevel=50e6  BaseVoltage=132e3  XRratio=7  BusType=PV  Pref=113e6  Qref=0  Prefabc=[10e3, 10e3, 10e3]  Qrefabc=[0, 0, 0]  Qmin=-inf  Qmax=inf
  Three-Phase Source26 : powerlib/Electrical Sources/Three-Phase Source  InternalConnection=Yg  VoltagePhases=off  Voltage=132e3  PhaseAngle=0  Voltage_phases=[25e3 25e3 25e3]/sqrt(3)  PhaseAngles_phases=[0 -120 +120]  Frequency=50  NonIdealSource=on  SpecifyImpedance=off  Resistance=0.8929  Inductance=16.58e-3  ShortCircuitLevel=50e6  BaseVoltage=132e3  XRratio=7  BusType=PV  Pref=113e6  Qref=0  Prefabc=[10e3, 10e3, 10e3]  Qrefabc=[0, 0, 0]  Qmin=-inf  Qmax=inf
  Three-Phase Source27 : powerlib/Electrical Sources/Three-Phase Source  InternalConnection=Yg  VoltagePhases=off  Voltage=230e3  PhaseAngle=0  Voltage_phases=[25e3 25e3 25e3]/sqrt(3)  PhaseAngles_phases=[0 -120 +120]  Frequency=50  NonIdealSource=on  SpecifyImpedance=off  Resistance=0.8929  Inductance=16.58e-3  ShortCircuitLevel=2e6  BaseVoltage=230e3  XRratio=7  BusType=PV  Pref=125e6  Qref=0  Prefabc=[10e3, 10e3, 10e3]  Qrefabc=[0, 0, 0]  Qmin=-100  Qmax=100
  Three-Phase Source28 : powerlib/Electrical Sources/Three-Phase Source  InternalConnection=Yg  VoltagePhases=off  Voltage=230e3  PhaseAngle=0  Voltage_phases=[25e3 25e3 25e3]/sqrt(3)  PhaseAngles_phases=[0 -120 +120]  Frequency=50  NonIdealSource=on  SpecifyImpedance=off  Resistance=0.8929  Inductance=16.58e-3  ShortCircuitLevel=2e6  BaseVoltage=230e3  XRratio=7  BusType=PV  Pref=125e6  Qref=0  Prefabc=[10e3, 10e3, 10e3]  Qrefabc=[0, 0, 0]  Qmin=-100  Qmax=100
  Three-Phase Source29 : powerlib/Electrical Sources/Three-Phase Source  InternalConnection=Yg  VoltagePhases=off  Voltage=230e3  PhaseAngle=0  Voltage_phases=[25e3 25e3 25e3]/sqrt(3)  PhaseAngles_phases=[0 -120 +120]  Frequency=50  NonIdealSource=on  SpecifyImpedance=off  Resistance=0.8929  Inductance=16.58e-3  ShortCircuitLevel=2e6  BaseVoltage=230e3  XRratio=7  BusType=PV  Pref=275e6  Qref=0  Prefabc=[10e3, 10e3, 10e3]  Qrefabc=[0, 0, 0]  Qmin=-100  Qmax=100
  Three-Phase Source3 : powerlib/Electrical Sources/Three-Phase Source  InternalConnection=Yg  VoltagePhases=off  Voltage=132e3  PhaseAngle=0  Voltage_phases=[25e3 25e3 25e3]/sqrt(3)  PhaseAngles_phases=[0 -120 +120]  Frequency=50  NonIdealSource=on  SpecifyImpedance=on  Resistance=0.8929  Inductance=16.58e-3  ShortCircuitLevel=50e6  BaseVoltage=132e3  XRratio=7  BusType=swing  Pref=113e6  Qref=0  Prefabc=[10e3, 10e3, 10e3]  Qrefabc=[0, 0, 0]  Qmin=-inf  Qmax=inf
  Three-Phase Source4 : powerlib/Electrical Sources/Three-Phase Source  InternalConnection=Yg  VoltagePhases=off  Voltage=132e3  PhaseAngle=0  Voltage_phases=[25e3 25e3 25e3]/sqrt(3)  PhaseAngles_phases=[0 -120 +120]  Frequency=50  NonIdealSource=on  SpecifyImpedance=off  Resistance=0.8929  Inductance=16.58e-3  ShortCircuitLevel=50e6  BaseVoltage=132e3  XRratio=7  BusType=PV  Pref=20e6  Qref=0  Prefabc=[10e3, 10e3, 10e3]  Qrefabc=[0, 0, 0]  Qmin=-inf  Qmax=inf
  Three-Phase Source5 : powerlib/Electrical Sources/Three-Phase Source  InternalConnection=Yg  VoltagePhases=off  Voltage=132e3  PhaseAngle=0  Voltage_phases=[25e3 25e3 25e3]/sqrt(3)  PhaseAngles_phases=[0 -120 +120]  Frequency=50  NonIdealSource=on  SpecifyImpedance=off  Resistance=0.8929  Inductance=16.58e-3  ShortCircuitLevel=50e6  BaseVoltage=132e3  XRratio=7  BusType=PV  Pref=21e6  Qref=0  Prefabc=[10e3, 10e3, 10e3]  Qrefabc=[0, 0, 0]  Qmin=-inf  Qmax=inf
  Three-Phase Source6 : powerlib/Electrical Sources/Three-Phase Source  InternalConnection=Yg  VoltagePhases=off  Voltage=132e3  PhaseAngle=0  Voltage_phases=[25e3 25e3 25e3]/sqrt(3)  PhaseAngles_phases=[0 -120 +120]  Frequency=50  NonIdealSource=on  SpecifyImpedance=off  Resistance=0.8929  Inductance=16.58e-3  ShortCircuitLevel=50e6  BaseVoltage=132e3  XRratio=7  BusType=PV  Pref=52e6  Qref=0  Prefabc=[10e3, 10e3, 10e3]  Qrefabc=[0, 0, 0]  Qmin=-inf  Qmax=inf
  Three-Phase Source7 : powerlib/Electrical Sources/Three-Phase Source  InternalConnection=Yg  VoltagePhases=off  Voltage=132e3  PhaseAngle=0  Voltage_phases=[25e3 25e3 25e3]/sqrt(3)  PhaseAngles_phases=[0 -120 +120]  Frequency=50  NonIdealSource=on  SpecifyImpedance=off  Resistance=0.8929  Inductance=16.58e-3  ShortCircuitLevel=50e6  BaseVoltage=132e3  XRratio=7  BusType=PV  Pref=50e6  Qref=0  Prefabc=[10e3, 10e3, 10e3]  Qrefabc=[0, 0, 0]  Qmin=-inf  Qmax=inf
  Three-Phase Source8 : powerlib/Electrical Sources/Three-Phase Source  InternalConnection=Yg  VoltagePhases=off  Voltage=132e3  PhaseAngle=0  Voltage_phases=[25e3 25e3 25e3]/sqrt(3)  PhaseAngles_phases=[0 -120 +120]  Frequency=50  NonIdealSource=on  SpecifyImpedance=off  Resistance=0.8929  Inductance=16.58e-3  ShortCircuitLevel=50e6  BaseVoltage=132e3  XRratio=7  BusType=PV  Pref=50e6  Qref=0  Prefabc=[10e3, 10e3, 10e3]  Qrefabc=[0, 0, 0]  Qmin=-inf  Qmax=inf
  Three-Phase Source9 : powerlib/Electrical Sources/Three-Phase Source  InternalConnection=Yg  VoltagePhases=off  Voltage=132e3  PhaseAngle=0  Voltage_phases=[25e3 25e3 25e3]/sqrt(3)  PhaseAngles_phases=[0 -120 +120]  Frequency=50  NonIdealSource=on  SpecifyImpedance=off  Resistance=0.8929  Inductance=16.58e-3  ShortCircuitLevel=50e6  BaseVoltage=132e3  XRratio=7  BusType=PV  Pref=50e6  Qref=0  Prefabc=[10e3, 10e3, 10e3]  Qrefabc=[0, 0, 0]  Qmin=-inf  Qmax=inf
  To Workspace : ToWorkspace  VariableName=voltage1  SaveFormat=Timeseries  SampleTime=-1
  To Workspace1 : ToWorkspace  VariableName=current1  SaveFormat=Timeseries  SampleTime=-1
  To Workspace2 : ToWorkspace  VariableName=voltage2  SaveFormat=Timeseries  SampleTime=-1
  To Workspace3 : ToWorkspace  VariableName=voltage3  SaveFormat=Timeseries  SampleTime=-1
  To Workspace4 : ToWorkspace  VariableName=current3  SaveFormat=Timeseries  SampleTime=-1
  To Workspace5 : ToWorkspace  VariableName=current2  SaveFormat=Timeseries  SampleTime=-1
  To Workspace6 : ToWorkspace  VariableName=voltage4  SaveFormat=Timeseries  SampleTime=-1
  To Workspace7 : ToWorkspace  VariableName=current4  SaveFormat=Timeseries  SampleTime=-1
  Voltage Measurement : powerlib/Measurements/Voltage Measurement  PhasorSimulation=off  OutputType=Complex  PSBequivalent=0
  powergui : powerlib/powergui  Priority=1  SimulationMode=Continuous  SampleTime=50e-6  frequency=60  Iterations=50  frequencyindice=60  Pbase=100e6  ErrMax=1e-4  UnitsV=kV  UnitsW=MW  buscounter=0  FunctionMessages=off  echomessages=off  EnableUseOfTLC=off  CurrentSourceSwitches=off  DisableSnubberDevices=off  DisableRonSwitches=off  DisableVfSwitches=off  DisplayEquations=off  AutomaticDiscreteSolvers=off  SolverType=Tustin/Backward Euler (TBE)  Interpol=off  ExternalGateDelay=off  methode=off  Ts=100  x0status=blocks  SPID=on  SwTol=0  HookPort=off  NonlinearTolerance=1e-4  nMaxIteration=100  ContinueOnMaxIteration=off  RestoreLinks=warning  ResistiveCurrentMeasurement=off  Frange=[0:2:500]  Ylog=off  Xlog=on  ShowGrid=off  save=off  variable=ZData  structure=0  ZoomFFT=off  StartTime=0.0  cycles=1  DisplayStyle=1  fundamental=60  FreqAxis=off  MaxFrequency=1000  frequencyindicesteady=1  RmsSteady=1  display=off
  wires:
  Palashbari/1 -> Demux/1
  Palashbari/2 -> Demux1/1
  Demux/1 -> Scope/1, To Workspace/1
  Demux1/1 -> Scope1/1, To Workspace1/1
  Demux/2 -> Scope/2, To Workspace2/1
  Demux/3 -> Scope/3, To Workspace3/1
  Demux1/3 -> Scope1/3, To Workspace4/1
  Demux1/2 -> Scope1/2, To Workspace5/1
  Voltage Measurement/1 -> Scope2/1, To Workspace6/1
  Current Measurement/1 -> Scope3/1, To Workspace7/1
  connections:
  Distributed Parameters Line/RConn2 -- Thakurgaon/LConn2
  Distributed Parameters Line/LConn2 -- Panchagarh/RConn2
  Distributed Parameters Line/LConn1 -- Panchagarh/RConn1
  Distributed Parameters Line/LConn3 -- Panchagarh/RConn3
  Distributed Parameters Line/RConn3 -- Thakurgaon/LConn3
  Distributed Parameters Line/RConn1 -- Thakurgaon/LConn1
  Thakurgaon/RConn2 -- Subsystem1/LConn2 -- Distributed Parameters Line1/LConn2 -- Distributed Parameters Line2/LConn2
  Distributed Parameters Line1/LConn3 -- Distributed Parameters Line2/LConn3 -- Subsystem1/LConn3 -- Thakurgaon/RConn3
  Purba Sadipur/LConn2 -- Distributed Parameters Line1/RConn2 -- Distributed Parameters Line2/RConn2
  Purba Sadipur/LConn3 -- Distributed Parameters Line2/RConn3 -- Distributed Parameters Line1/RConn3
  Purba Sadipur/LConn1 -- Distributed Parameters Line1/RConn1 -- Distributed Parameters Line2/RConn1
  Distributed Parameters Line3/RConn1 -- Distributed Parameters Line4/RConn1 -- Distributed Parameters Line7/RConn1 -- Distributed Parameters Line8/RConn1 -- Saidpur/LConn1
  Distributed Parameters Line3/RConn2 -- Distributed Parameters Line7/RConn2 -- Distributed Parameters Line8/RConn2 -- Saidpur/LConn2 -- Distributed Parameters Line4/RConn2
  Distributed Parameters Line3/RConn3 -- Distributed Parameters Line7/RConn3 -- Distributed Parameters Line8/RConn3 -- Saidpur/LConn3 -- Distributed Parameters Line4/RConn3
  Distributed Parameters Line3/LConn1 -- Distributed Parameters Line4/LConn1 -- Subsystem2/LConn1 -- Purba Sadipur/RConn1
  Distributed Parameters Line3/LConn3 -- Subsystem2/LConn3 -- Purba Sadipur/RConn3 -- Distributed Parameters Line4/LConn3
  Distributed Parameters Line3/LConn2 -- Distributed Parameters Line4/LConn2 -- Subsystem2/LConn2 -- Purba Sadipur/RConn2
  Subsystem4/LConn2 -- Three-Phase Source/RConn2 -- Saidpur/RConn2 -- Distributed Parameters Line5/LConn2 -- Distributed Parameters Line10/LConn2 -- Distributed Parameters Line9/LConn2 -- Distributed Parameters Line6/LConn2
  Distributed Parameters Line5/RConn2 -- Distributed Parameters Line6/RConn2 -- Rangpur/LConn2
  Distributed Parameters Line10/LConn1 -- Distributed Parameters Line9/LConn1 -- Distributed Parameters Line5/LConn1 -- Distributed Parameters Line6/LConn1 -- Subsystem4/LConn1 -- Saidpur/RConn1 -- Three-Phase Source/RConn1
  Distributed Parameters Line5/RConn1 -- Distributed Parameters Line6/RConn1 -- Rangpur/LConn1
  Distributed Parameters Line5/RConn3 -- Distributed Parameters Line6/RConn3 -- Rangpur/LConn3
  Distributed Parameters Line8/LConn1 -- Distributed Parameters Line7/LConn1 -- Jaldhaka/RConn1
  Distributed Parameters Line8/LConn2 -- Distributed Parameters Line7/LConn2 -- Jaldhaka/RConn2
  Distributed Parameters Line8/LConn3 -- Distributed Parameters Line7/LConn3 -- Jaldhaka/RConn3
  Distributed Parameters Line9/RConn1 -- Distributed Parameters Line10/RConn1 -- Distributed Parameters Line12/RConn1 -- Distributed Parameters Line11/RConn1 -- Barapukuria/LConn1
  Distributed Parameters Line9/RConn2 -- Distributed Parameters Line10/RConn2 -- Distributed Parameters Line12/RConn2 -- Distributed Parameters Line11/RConn2 -- Barapukuria/LConn2
  Distributed Parameters Line9/RConn3 -- Distributed Parameters Line10/RConn3 -- Distributed Parameters Line12/RConn3 -- Distributed Parameters Line11/RConn3 -- Barapukuria/LConn3
  Distributed Parameters Line12/LConn1 -- Distributed Parameters Line11/LConn1 -- Distributed Parameters Line16/LConn1 -- Distributed Parameters Line15/LConn1 -- Distributed Parameters Line14/LConn1 -- Distributed Parameters Line13/LConn1 -- Three-Phase Source1/RConn1 -- Subsystem6/LConn3 -- Rangpur/RConn1
  Distributed Parameters Line12/LConn2 -- Distributed Parameters Line11/LConn2 -- Distributed Parameters Line16/LConn2 -- Distributed Parameters Line15/LConn2 -- Distributed Parameters Line14/LConn2 -- Distributed Parameters Line13/LConn2 -- Subsystem6/LConn2 -- Three-Phase Source1/RConn2 -- Rangpur/RConn2
  Kurigram/LConn1 -- Distributed Parameters Line13/RConn1
  Distributed Parameters Line13/RConn2 -- Kurigram/LConn2
  Distributed Parameters Line13/RConn3 -- Kurigram/LConn3
  Distributed Parameters Line14/RConn2 -- Lalmonirhat/LConn2
  Lalmonirhat/LConn1 -- Distributed Parameters Line14/RConn1
  Distributed Parameters Line14/RConn3 -- Lalmonirhat/LConn3
  Palashbari/LConn2 -- Distributed Parameters Line16/RConn2 -- Distributed Parameters Line15/RConn2
  Palashbari/LConn1 -- Distributed Parameters Line16/RConn1 -- Distributed Parameters Line15/RConn1
  Palashbari/LConn3 -- Distributed Parameters Line16/RConn3 -- Distributed Parameters Line15/RConn3
  Palashbari/RConn1 -- Three-Phase Source2/RConn1 -- Subsystem9/LConn1 -- Three-Phase Fault/LConn1 -- Distributed Parameters Line18/LConn1 -- Distributed Parameters Line17/LConn1
  Three-Phase Source2/RConn3 -- Subsystem9/LConn3 -- Three-Phase Fault/LConn3 -- Distributed Parameters Line17/LConn3 -- Distributed Parameters Line18/LConn3 -- Palashbari/RConn3
  Mahastangarh/LConn2 -- Distributed Parameters Line18/RConn2 -- Distributed Parameters Line17/RConn2
  Distributed Parameters Line18/RConn1 -- Distributed Parameters Line17/RConn1 -- Mahastangarh/LConn1
  Mahastangarh/LConn3 -- Distributed Parameters Line18/RConn3 -- Distributed Parameters Line17/RConn3
  Distributed Parameters Line19/LConn1 -- Distributed Parameters Line20/LConn1 -- Subsystem10/LConn1 -- Mahastangarh/RConn1
  Distributed Parameters Line20/LConn2 -- Distributed Parameters Line19/LConn2 -- Subsystem10/LConn2 -- Mahastangarh/RConn2
  Mahastangarh/RConn3 -- Distributed Parameters Line20/LConn3 -- Distributed Parameters Line19/LConn3 -- Subsystem10/LConn3
  Distributed Parameters Line19/RConn2 -- Distributed Parameters Line20/RConn2 -- Distributed Parameters Line21/RConn2 -- Distributed Parameters Line22/RConn2 -- Bogura/LConn2
  Distributed Parameters Line19/RConn3 -- Distributed Parameters Line20/RConn3 -- Distributed Parameters Line22/RConn3 -- Distributed Parameters Line21/RConn3 -- Bogura/LConn3
  Distributed Parameters Line19/RConn1 -- Distributed Parameters Line20/RConn1 -- Distributed Parameters Line22/RConn1 -- Distributed Parameters Line21/RConn1 -- Bogura/LConn1
  Distributed Parameters Line21/LConn1 -- Distributed Parameters Line22/LConn1 -- Three-Phase Source3/RConn1 -- Subsystem13/LConn1 -- Naogaon/RConn1
  Distributed Parameters Line21/LConn2 -- Distributed Parameters Line22/LConn2 -- Subsystem13/LConn2 -- Three-Phase Source3/RConn2 -- Naogaon/RConn2
  Distributed Parameters Line21/LConn3 -- Distributed Parameters Line22/LConn3 -- Subsystem13/LConn3 -- Three-Phase Source3/RConn3 -- Naogaon/RConn3
  Distributed Parameters Line23/RConn2 -- Distributed Parameters Line24/RConn2 -- Naogaon/LConn2
  Distributed Parameters Line23/RConn1 -- Naogaon/LConn1 -- Distributed Parameters Line24/RConn1
  Distributed Parameters Line23/RConn3 -- Distributed Parameters Line24/RConn3 -- Naogaon/LConn3
  Distributed Parameters Line24/LConn3 -- Niyamotpur/LConn3
  Three-Phase Source26/RConn1 -- Three-Phase Source25/RConn1 -- Three-Phase Transformer (Two Windings)91/RConn1 -- Three-Phase Transformer (Two Windings)89/RConn1 -- Three-Phase Transformer (Two Windings)90/RConn1 -- Bogura New/RConn1
  Three-Phase Source26/RConn2 -- Three-Phase Source25/RConn2 -- Three-Phase Transformer (Two Windings)89/RConn2 -- Three-Phase Transformer (Two Windings)91/RConn2 -- Three-Phase Transformer (Two Windings)90/RConn2 -- Bogura New/RConn2
  Three-Phase Source26/RConn3 -- Three-Phase Source25/RConn3 -- Three-Phase Transformer (Two Windings)91/RConn3 -- Three-Phase Transformer (Two Windings)89/RConn3 -- Three-Phase Transformer (Two Windings)90/RConn3 -- Bogura New/RConn3
  Distributed Parameters Line25/LConn3 -- Distributed Parameters Line26/LConn3 -- Three-Phase Source5/RConn3 -- Three-Phase Source4/RConn3 -- Distributed Parameters Line28/LConn3 -- Distributed Parameters Line27/LConn3 -- Bogura/RConn3 -- Subsystem18/LConn3
  Bogura New/LConn2 -- Distributed Parameters Line42/LConn2 -- Distributed Parameters Line43/LConn2 -- Distributed Parameters Line26/RConn2 -- Distributed Parameters Line25/RConn2
  Bogura New/LConn1 -- Distributed Parameters Line42/LConn1 -- Distributed Parameters Line43/LConn1 -- Distributed Parameters Line26/RConn1 -- Distributed Parameters Line25/RConn1
  Distributed Parameters Line25/RConn3 -- Distributed Parameters Line26/RConn3 -- Distributed Parameters Line42/LConn3 -- Distributed Parameters Line43/LConn3 -- Bogura New/LConn3
  Distributed Parameters Line27/RConn2 -- Distributed Parameters Line28/RConn2 -- Natore/LConn2
  Natore/LConn1 -- Distributed Parameters Line28/RConn1 -- Distributed Parameters Line27/RConn1
  Natore/LConn3 -- Distributed Parameters Line28/RConn3 -- Distributed Parameters Line27/RConn3
  Distributed Parameters Line29/RConn2 -- Distributed Parameters Line30/RConn2 -- Ishwardi/LConn2
  Distributed Parameters Line29/RConn1 -- Distributed Parameters Line30/RConn1 -- Ishwardi/LConn1
  Distributed Parameters Line29/RConn3 -- Distributed Parameters Line30/RConn3 -- Ishwardi/LConn3
  Distributed Parameters Line29/LConn2 -- Distributed Parameters Line32/RConn2 -- Distributed Parameters Line31/RConn2 -- Three-Phase Source6/RConn2 -- Subsystem20/LConn2 -- Natore/RConn2 -- Distributed Parameters Line30/LConn2
  Distributed Parameters Line29/LConn1 -- Distributed Parameters Line30/LConn1 -- Distributed Parameters Line32/RConn1 -- Distributed Parameters Line31/RConn1 -- Natore/RConn1 -- Three-Phase Source6/RConn1 -- Subsystem20/LConn1
  Distributed Parameters Line31/LConn1 -- Distributed Parameters Line32/LConn1 -- Subsystem17/LConn1 -- Three-Phase Source8/RConn1 -- Three-Phase Source7/RConn1 -- Rajshahi/RConn1
  Distributed Parameters Line31/LConn2 -- Distributed Parameters Line32/LConn2 -- Subsystem17/LConn2 -- Three-Phase Source8/RConn2 -- Three-Phase Source7/RConn2 -- Rajshahi/RConn2
  Distributed Parameters Line31/LConn3 -- Distributed Parameters Line32/LConn3 -- Subsystem17/LConn3 -- Three-Phase Source8/RConn3 -- Three-Phase Source7/RConn3 -- Rajshahi/RConn3
  Distributed Parameters Line33/RConn2 -- Distributed Parameters Line34/RConn2 -- Rajshahi/LConn2
  Distributed Parameters Line33/LConn1 -- Distributed Parameters Line36/RConn1 -- Distributed Parameters Line35/RConn1 -- Rajshahi (N)/RConn1 -- Distributed Parameters Line34/LConn1
  Distributed Parameters Line33/RConn1 -- Distributed Parameters Line34/RConn1 -- Rajshahi/LConn1
  Distributed Parameters Line33/RConn3 -- Rajshahi/LConn3 -- Distributed Parameters Line34/RConn3
  Distributed Parameters Line33/LConn3 -- Distributed Parameters Line35/RConn3 -- Rajshahi (N)/RConn3 -- Distributed Parameters Line34/LConn3 -- Distributed Parameters Line36/RConn3
  Chapai Nawabganj/LConn1 -- Distributed Parameters Line37/LConn1 -- Distributed Parameters Line35/LConn1
  Chapai Nawabganj/LConn2 -- Distributed Parameters Line37/LConn2 -- Distributed Parameters Line35/LConn2
  Chapai Nawabganj/LConn3 -- Distributed Parameters Line35/LConn3 -- Distributed Parameters Line37/LConn3
  Amnura/LConn2 -- Distributed Parameters Line37/RConn2 -- Distributed Parameters Line36/LConn2
  Distributed Parameters Line36/LConn1 -- Amnura/LConn1 -- Distributed Parameters Line37/RConn3
  Distributed Parameters Line36/LConn3 -- Distributed Parameters Line37/RConn1 -- Amnura/LConn3
  Three-Phase Source10/RConn2 -- Three-Phase Source9/RConn2 -- Subsystem16/LConn2 -- Amnura/RConn2
  Three-Phase Source10/RConn1 -- Three-Phase Source9/RConn1 -- Subsystem16/LConn1 -- Amnura/RConn3
  Three-Phase Source10/RConn3 -- Three-Phase Source9/RConn3 -- Subsystem16/LConn3 -- Amnura/RConn1
  Rooppur/LConn3 -- Distributed Parameters Line38/LConn3
  Distributed Parameters Line38/LConn2 -- Rooppur/LConn2
  Distributed Parameters Line38/LConn1 -- Rooppur/LConn1
  Distributed Parameters Line38/RConn1 -- Three-Phase Transformer (Two Windings)96/RConn1 -- Three-Phase Transformer (Two Windings)95/RConn1 -- Three-Phase Transformer (Two Windings)94/RConn1 -- Distributed Parameters Line40/LConn1 -- Distributed Parameters Line39/LConn1 -- Distributed Parameters Line41/LConn1 -- Distributed Parameters Line47/LConn1 -- Subsystem22/LConn1 -- Series RLC Branch/LConn1 -- Ishwardi/RConn1
  Distributed Parameters Line38/RConn2 -- Three-Phase Transformer (Two Windings)96/RConn2 -- Three-Phase Transformer (Two Windings)95/RConn2 -- Three-Phase Transformer (Two Windings)94/RConn2 -- Distributed Parameters Line39/LConn2 -- Distributed Parameters Line40/LConn2 -- Distributed Parameters Line41/LConn2 -- Distributed Parameters Line47/LConn2 -- Subsystem22/LConn2 -- Ishwardi/RConn2 -- Series RLC Branch1/LConn1
  Distributed Parameters Line38/RConn3 -- Three-Phase Transformer (Two Windings)96/RConn3 -- Three-Phase Transformer (Two Windings)95/RConn3 -- Three-Phase Transformer (Two Windings)94/RConn3 -- Distributed Parameters Line40/LConn3 -- Distributed Parameters Line39/LConn3 -- Distributed Parameters Line41/LConn3 -- Distributed Parameters Line47/LConn3 -- Subsystem22/LConn3 -- Ishwardi/RConn3 -- Series RLC Branch2/LConn1
  Distributed Parameters Line39/RConn2 -- Bheramara/LConn2 -- Distributed Parameters Line40/RConn2
  Bheramara/LConn1 -- Distributed Parameters Line40/RConn1 -- Distributed Parameters Line39/RConn1
  Bheramara/LConn3 -- Distributed Parameters Line40/RConn3 -- Distributed Parameters Line39/RConn3
  Three-Phase Source19/RConn2 -- Three-Phase Source18/RConn2 -- Three-Phase Source17/RConn2 -- Three-Phase Source16/RConn2 -- Subsystem26/RConn2 -- Bheramara/RConn2
  Three-Phase Source19/RConn1 -- Three-Phase Source18/RConn1 -- Subsystem26/RConn3 -- Bheramara/RConn1 -- Three-Phase Source16/RConn1 -- Three-Phase Source17/RConn1
  Distributed Parameters Line41/RConn1 -- Baghabari/LConn1
  Distributed Parameters Line41/RConn2 -- Baghabari/LConn2
  Distributed Parameters Line41/RConn3 -- Baghabari/LConn3
  Three-Phase Source13/RConn1 -- Three-Phase Source12/RConn1 -- Three-Phase Transformer (Two Windings)93/RConn1 -- Three-Phase Transformer (Two Windings)92/RConn1 -- Distributed Parameters Line50/LConn1 -- Distributed Parameters Line49/LConn1 -- Distributed Parameters Line51/RConn1 -- Baghabari/RConn1 -- Three-Phase Source11/RConn1 -- Three-Phase Source14/RConn1
  Three-Phase Source14/RConn2 -- Three-Phase Source12/RConn2 -- Three-Phase Transformer (Two Windings)93/RConn2 -- Three-Phase Transformer (Two Windings)92/RConn2 -- Distributed Parameters Line50/LConn2 -- Distributed Parameters Line49/LConn2 -- Distributed Parameters Line51/RConn2 -- Baghabari/RConn2 -- Three-Phase Source11/RConn2 -- Three-Phase Source13/RConn2
  Three-Phase Source11/RConn3 -- Three-Phase Source14/RConn3 -- Three-Phase Source13/RConn3 -- Three-Phase Source12/RConn3 -- Three-Phase Transformer (Two Windings)93/RConn3 -- Three-Phase Transformer (Two Windings)92/RConn3 -- Distributed Parameters Line50/LConn3 -- Distributed Parameters Line49/LConn3 -- Distributed Parameters Line51/RConn3 -- Baghabari/RConn3
  Distributed Parameters Line42/RConn2 -- Sherpur (B)/LConn2 -- Distributed Parameters Line43/RConn2
  Distributed Parameters Line42/RConn1 -- Distributed Parameters Line43/RConn1 -- Sherpur (B)/LConn1
  Distributed Parameters Line42/RConn3 -- Distributed Parameters Line43/RConn3 -- Sherpur (B)/LConn3
  Distributed Parameters Line44/RConn2 -- Distributed Parameters Line45/RConn2 -- Sirajganj/LConn2
  Distributed Parameters Line44/LConn1 -- Distributed Parameters Line45/LConn1 -- Subsystem19/LConn1 -- Sherpur (B)/RConn1
  Distributed Parameters Line44/LConn3 -- Distributed Parameters Line45/LConn3 -- Subsystem19/LConn3 -- Sherpur (B)/RConn3
  Distributed Parameters Line44/RConn3 -- Distributed Parameters Line45/RConn3 -- Sirajganj/LConn3
  Distributed Parameters Line44/RConn1 -- Distributed Parameters Line45/RConn1 -- Sirajganj/LConn1
  Distributed Parameters Line46/RConn2 -- Shahjadpur/LConn2
  Distributed Parameters Line46/RConn1 -- Shahjadpur/LConn1
  Shahjadpur/LConn3 -- Distributed Parameters Line46/RConn3
  Distributed Parameters Line46/LConn3 -- Sirajganj/RConn3 -- Subsystem23/LConn3 -- Distributed Parameters Line51/LConn3
  Distributed Parameters Line46/LConn1 -- Sirajganj/RConn1 -- Subsystem23/LConn1 -- Distributed Parameters Line51/LConn1
  Pabna/LConn1 -- Subsystem25/LConn1 -- Distributed Parameters Line47/RConn1
  Distributed Parameters Line48/LConn2 -- Pabna/RConn2
  Distributed Parameters Line48/LConn1 -- Pabna/RConn1
  Distributed Parameters Line48/LConn3 -- Pabna/RConn3
  Distributed Parameters Line48/RConn2 -- Distributed Parameters Line50/RConn2 -- Distributed Parameters Line49/RConn2 -- Shahjadpur/RConn2 -- Subsystem24/RConn2 -- Three-Phase Source15/RConn2
  Three-Phase Source20/RConn2 -- Baghabari PP/RConn2 -- Distributed Parameters Line55/RConn2 -- Distributed Parameters Line54/RConn2
  Three-Phase Source20/RConn1 -- Baghabari PP/RConn1 -- Distributed Parameters Line55/RConn1 -- Distributed Parameters Line54/RConn1
  Three-Phase Source20/RConn3 -- Baghabari PP/RConn3 -- Distributed Parameters Line55/RConn3 -- Distributed Parameters Line54/RConn3
  Ishwardi PP/RConn1 -- Distributed Parameters Line53/LConn1 -- Distributed Parameters Line52/LConn1
  Distributed Parameters Line52/LConn2 -- Distributed Parameters Line53/LConn2 -- Ishwardi PP/RConn2
  Distributed Parameters Line52/LConn3 -- Distributed Parameters Line53/LConn3 -- Ishwardi PP/RConn3
  Distributed Parameters Line54/LConn2 -- Distributed Parameters Line55/LConn2 -- Three-Phase Source24/RConn2 -- Three-Phase Source22/RConn2 -- Three-Phase Source23/RConn2 -- Three-Phase Source21/RConn2 -- Sirajganj SW PP/RConn2
  Distributed Parameters Line54/LConn1 -- Distributed Parameters Line55/LConn1 -- Three-Phase Source24/RConn1 -- Three-Phase Source23/RConn1 -- Three-Phase Source22/RConn1 -- Three-Phase Source21/RConn1 -- Sirajganj SW PP/RConn1
  Distributed Parameters Line54/LConn3 -- Distributed Parameters Line55/LConn3 -- Three-Phase Source24/RConn3 -- Three-Phase Source23/RConn3 -- Three-Phase Source22/RConn3 -- Three-Phase Source21/RConn3 -- Sirajganj SW PP/RConn3
  Distributed Parameters Line56/RConn2 -- Distributed Parameters Line57/RConn2 -- Sirajganj SW PP/LConn2
  Distributed Parameters Line56/RConn1 -- Distributed Parameters Line57/RConn1 -- Sirajganj SW PP/LConn1
  Distributed Parameters Line56/RConn3 -- Distributed Parameters Line57/RConn3 -- Sirajganj SW PP/LConn3
  Distributed Parameters Line56/LConn1 -- Distributed Parameters Line59/RConn1 -- Distributed Parameters Line58/RConn1 -- Bogura New PP/RConn1 -- Distributed Parameters Line57/LConn1
  Distributed Parameters Line56/LConn2 -- Distributed Parameters Line59/RConn2 -- Distributed Parameters Line58/RConn2 -- Bogura New PP/RConn2 -- Distributed Parameters Line57/LConn2
  Distributed Parameters Line56/LConn3 -- Distributed Parameters Line59/RConn3 -- Distributed Parameters Line58/RConn3 -- Bogura New PP/RConn3 -- Distributed Parameters Line57/LConn3
  Barapukuria PP/RConn1 -- Distributed Parameters Line59/LConn1 -- Distributed Parameters Line58/LConn1 -- Three-Phase Source27/RConn1 -- Three-Phase Source29/RConn1 -- Three-Phase Source28/RConn1
  Distributed Parameters Line58/LConn2 -- Three-Phase Source29/RConn2 -- Three-Phase Source28/RConn2 -- Barapukuria PP/RConn2 -- Three-Phase Source27/RConn2 -- Distributed Parameters Line59/LConn2
  Distributed Parameters Line58/LConn3 -- Three-Phase Source29/RConn3 -- Three-Phase Source28/RConn3 -- Barapukuria PP/RConn3 -- Three-Phase Source27/RConn3 -- Distributed Parameters Line59/LConn3
  Ground/LConn1 -- Series RLC Branch2/RConn1 -- Series RLC Branch1/RConn1 -- Series RLC Branch/RConn1
  Three-Phase Transformer (Two Windings)86/LConn2 -- Three-Phase Transformer (Two Windings)87/LConn2 -- Barapukuria PP/LConn2 -- Three-Phase Transformer (Two Windings)88/LConn2
  Three-Phase Transformer (Two Windings)86/LConn1 -- Three-Phase Transformer (Two Windings)88/LConn1 -- Barapukuria PP/LConn1 -- Three-Phase Transformer (Two Windings)87/LConn1
  Barapukuria PP/LConn3 -- Three-Phase Transformer (Two Windings)88/LConn3 -- Three-Phase Transformer (Two Windings)86/LConn3 -- Three-Phase Transformer (Two Windings)87/LConn3
  Three-Phase Transformer (Two Windings)90/LConn2 -- Three-Phase Transformer (Two Windings)91/LConn2 -- Three-Phase Transformer (Two Windings)89/LConn2 -- Bogura New PP/LConn2
  Three-Phase Transformer (Two Windings)90/LConn1 -- Three-Phase Transformer (Two Windings)91/LConn1 -- Three-Phase Transformer (Two Windings)89/LConn1 -- Bogura New PP/LConn1
  Three-Phase Transformer (Two Windings)90/LConn3 -- Three-Phase Transformer (Two Windings)91/LConn3 -- Three-Phase Transformer (Two Windings)89/LConn3 -- Bogura New PP/LConn3
  Distributed Parameters Line53/RConn3 -- Distributed Parameters Line52/RConn3 -- Three-Phase Transformer (Two Windings)93/LConn3 -- Three-Phase Transformer (Two Windings)92/LConn3 -- Baghabari PP/LConn3
  Distributed Parameters Line53/RConn2 -- Distributed Parameters Line52/RConn2 -- Three-Phase Transformer (Two Windings)93/LConn2 -- Three-Phase Transformer (Two Windings)92/LConn2 -- Baghabari PP/LConn2
  Distributed Parameters Line53/RConn1 -- Distributed Parameters Line52/RConn1 -- Three-Phase Transformer (Two Windings)93/LConn1 -- Three-Phase Transformer (Two Windings)92/LConn1 -- Baghabari PP/LConn1
  Three-Phase Transformer (Two Windings)94/LConn1 -- Three-Phase Transformer (Two Windings)96/LConn1 -- Three-Phase Transformer (Two Windings)95/LConn1 -- Ishwardi PP/LConn1
  Ishwardi PP/LConn2 -- Three-Phase Transformer (Two Windings)96/LConn2 -- Three-Phase Transformer (Two Windings)95/LConn2 -- Three-Phase Transformer (Two Windings)94/LConn2
  Ishwardi PP/LConn3 -- Three-Phase Transformer (Two Windings)96/LConn3 -- Three-Phase Transformer (Two Windings)95/LConn3 -- Three-Phase Transformer (Two Windings)94/LConn3
  Distributed Parameters Line33/LConn2 -- Distributed Parameters Line36/RConn2 -- Distributed Parameters Line35/RConn2 -- Rajshahi (N)/RConn2 -- Distributed Parameters Line34/LConn2
  Panchagarh/LConn3 -- Subsystem/LConn1
  Subsystem/LConn2 -- Panchagarh/LConn2
  Panchagarh/LConn1 -- Subsystem/LConn3
  Distributed Parameters Line2/LConn1 -- Distributed Parameters Line1/LConn1 -- Subsystem1/LConn1 -- Thakurgaon/RConn1
  Subsystem3/LConn1 -- Jaldhaka/LConn3
  Subsystem3/LConn2 -- Jaldhaka/LConn2
  Subsystem3/LConn3 -- Jaldhaka/LConn1
  Distributed Parameters Line6/LConn3 -- Subsystem4/LConn3 -- Three-Phase Source/RConn3 -- Saidpur/RConn3 -- Distributed Parameters Line10/LConn3 -- Distributed Parameters Line9/LConn3 -- Distributed Parameters Line5/LConn3
  Three-Phase Transformer (Two Windings)88/RConn1 -- Three-Phase Transformer (Two Windings)87/RConn1 -- Three-Phase Transformer (Two Windings)86/RConn1 -- Subsystem5/LConn2 -- Barapukuria/RConn1
  Three-Phase Transformer (Two Windings)86/RConn3 -- Three-Phase Transformer (Two Windings)87/RConn3 -- Subsystem5/LConn4 -- Barapukuria/RConn3 -- Three-Phase Transformer (Two Windings)88/RConn3
  Three-Phase Transformer (Two Windings)87/RConn2 -- Three-Phase Transformer (Two Windings)86/RConn2 -- Three-Phase Transformer (Two Windings)88/RConn2 -- Subsystem5/LConn3 -- Barapukuria/RConn2
  Three-Phase Source1/RConn3 -- Distributed Parameters Line12/LConn3 -- Distributed Parameters Line11/LConn3 -- Distributed Parameters Line16/LConn3 -- Distributed Parameters Line14/LConn3 -- Distributed Parameters Line15/LConn3 -- Distributed Parameters Line13/LConn3 -- Rangpur/RConn3 -- Subsystem6/LConn1
  Subsystem7/LConn1 -- Kurigram/RConn1
  Subsystem7/LConn2 -- Kurigram/RConn2
  Subsystem7/LConn3 -- Kurigram/RConn3
  Subsystem8/LConn1 -- Lalmonirhat/RConn1
  Subsystem8/LConn2 -- Lalmonirhat/RConn2
  Subsystem8/LConn3 -- Lalmonirhat/RConn3
  Three-Phase Source2/RConn2 -- Subsystem9/LConn2 -- Three-Phase Fault/LConn2 -- Distributed Parameters Line17/LConn2 -- Distributed Parameters Line18/LConn2 -- Palashbari/RConn2
  Distributed Parameters Line23/LConn1 -- Joypurhat/RConn1
  Distributed Parameters Line23/LConn2 -- Joypurhat/RConn2
  Distributed Parameters Line23/LConn3 -- Joypurhat/RConn3
  Joypurhat/LConn3 -- Subsystem11/LConn1
  Joypurhat/LConn2 -- Subsystem11/LConn2
  Joypurhat/LConn1 -- Subsystem11/LConn3
  Distributed Parameters Line24/LConn2 -- Niyamotpur/LConn2
  Distributed Parameters Line24/LConn1 -- Niyamotpur/LConn1
  Subsystem12/LConn1 -- Niyamotpur/RConn1
  Subsystem12/LConn2 -- Niyamotpur/RConn2
  Subsystem12/LConn3 -- Niyamotpur/RConn3
  Subsystem14/LConn1 -- Chapai Nawabganj/RConn3
  Subsystem14/LConn2 -- Chapai Nawabganj/RConn2
  Subsystem14/LConn3 -- Chapai Nawabganj/RConn1
  Subsystem15/LConn1 -- Rajshahi (N)/LConn3
  Subsystem15/LConn2 -- Rajshahi (N)/LConn2
  Subsystem15/LConn3 -- Rajshahi (N)/LConn1
  Three-Phase Source5/RConn2 -- Three-Phase Source4/RConn2 -- Distributed Parameters Line25/LConn2 -- Distributed Parameters Line26/LConn2 -- Distributed Parameters Line28/LConn2 -- Distributed Parameters Line27/LConn2 -- Bogura/RConn2 -- Subsystem18/LConn2
  Distributed Parameters Line28/LConn1 -- Three-Phase Source5/RConn1 -- Three-Phase Source4/RConn1 -- Distributed Parameters Line25/LConn1 -- Distributed Parameters Line26/LConn1 -- Subsystem18/LConn1 -- Bogura/RConn1 -- Distributed Parameters Line27/LConn1
  Sherpur (B)/RConn2 -- Subsystem19/LConn2 -- Distributed Parameters Line45/LConn2 -- Distributed Parameters Line44/LConn2
  Distributed Parameters Line29/LConn3 -- Distributed Parameters Line30/LConn3 -- Distributed Parameters Line32/RConn3 -- Distributed Parameters Line31/RConn3 -- Natore/RConn3 -- Three-Phase Source6/RConn3 -- Subsystem20/LConn3
  Subsystem21/RConn1 -- Rooppur/RConn1
  Subsystem21/RConn2 -- Rooppur/RConn2
  Subsystem21/RConn3 -- Rooppur/RConn3
  Distributed Parameters Line46/LConn2 -- Sirajganj/RConn2 -- Subsystem23/LConn2 -- Distributed Parameters Line51/LConn2
  Distributed Parameters Line48/RConn3 -- Distributed Parameters Line50/RConn3 -- Distributed Parameters Line49/RConn3 -- Shahjadpur/RConn3 -- Subsystem24/RConn3 -- Three-Phase Source15/RConn3
  Distributed Parameters Line48/RConn1 -- Distributed Parameters Line50/RConn1 -- Distributed Parameters Line49/RConn1 -- Subsystem24/RConn1 -- Three-Phase Source15/RConn1 -- Shahjadpur/RConn1
  Distributed Parameters Line47/RConn2 -- Pabna/LConn2 -- Subsystem25/LConn2
  Distributed Parameters Line47/RConn3 -- Pabna/LConn3 -- Subsystem25/LConn3
  Three-Phase Source19/RConn3 -- Subsystem26/RConn1 -- Bheramara/RConn3 -- Three-Phase Source16/RConn3 -- Three-Phase Source17/RConn3 -- Three-Phase Source18/RConn3
  Three-Phase Source2/LConn1 -- Voltage Measurement/LConn1 -- Current Measurement/LConn1
  Voltage Measurement/LConn2 -- Current Measurement/RConn1 -- Ground1/LConn1
